simulink model "test"  (R2025b)
settings: Solver=FixedStepDiscrete  StartTime=0.0  StopTime=10.0  FixedStep=0.001  RelTol=1e-3
undefined symbols (not defined in the file): QFN64, SAMC21J18A, Timer
libraries: MCHP_Blockset x3
settings Model: SimulationMode=external  Creator=maxbo  LastModifiedBy=maxbo
settings OptimizationCC: DefaultParameterBehavior=Inlined  EnhancedBackFolding=on  PassReuseOutputArgsAs=Individual arguments  ZeroExternalMemoryAtStartup=off  ZeroInternalMemoryAtStartup=off  OptimizeBlockOrder=speed  DifferentSizesBufferReuse=on  OptimizationCustomize=off  EfficientTunableParamExpr=on
settings DebuggingCC: ParameterTunabilityLossMsg=error
settings SFSimCC: MATLABDynamicMemAlloc=off
settings RTWCC: SystemTargetFile=MCHP_ARM7_stf.tlc  TemplateMakefile=MCHP_ARM7.tmf  Toolchain=MPLAB XC32 - v5.10 for SAM & PIC32 MCUs (Microchip)  BuildConfiguration=Specify  Description=Microchip Embedded Target Cortex M7 (real-time)
settings CodeAppCC: ForceParamTrailComments=on  IgnoreCustomStorageClasses=off  OperatorAnnotations=on  SimulinkDataObjDesc=on  SFDataObjDesc=on  InsertBlockDesc=on
settings STFCustomTargetCC: SystemTargetFile=MCHP_ARM7_stf.tlc  TargetLangStandard=C99 (ISO)  MultiwordLength=256.0  ConcurrentExecutionCompliant=off  IncludeMdlTerminateFcn=off  CombineOutputUpdateFcns=on  ERTCustomFileBanners=on  SupportContinuousTime=off  RemoveResetFunc=on  MATLABClassNameForMDSCustomization=Simulink.SoftwareTarget.ERTCustomization  GRTInterface=off  BIN2HEX=xc32-bin2hex  TIMER_PRESCALER=[0 -1 -1 -1 -1]  MCHP_AUTO_FLASH=off  AssemblyListing=off  TIMER_START=[1]  PIC_REF=SAMC21J18A  RTWGenSettings_txt="s.MIPS='48000000';s.VDD_RANGE='5';s.QUARTZ='48000000';s.PLL_ENABLED='0';s.MIPS_DESIRED='48000000';s.MCLK_CPUDIV='1';s.CPU_SRC='0';s.GCLK_PCHCTRLn='[-1 -1 -1 -1 -1 -1 -1 -1 -1 -1 -1 -1 -1 -1 -1 -1 -1 -1 -1 -1 -1 -1 -1 -1 -1 -1 -1 -1 -1 -1 -1 -1 -1 -1 -1 -1 -1 -1 -1 -1 -1 -1 -1 -1 -1 -1 -1 -1]';s.OSC32KCTRL_XOSC32K_CONFIG='0';s.OSC32KCTRL_XOSC32K_ENABLE='0';s.OSC32KCTRL_XOSC32K_STARTUP='2';s.OSC32KCTRL_XOSC32K_ONDEMAND='0';s.OSC32KCTRL_XOSC32K_RUNSTDBY='1';s.OSC32KCTRL_XOSC32K_EN1K='0';s.OSC32KCTRL_XOSC32K_EN32K='1';s.OSC32KCTRL_XOSC32K_XTALEN='0';s.OSC32KCTRL_OSC32K_CONFIG='0';s.OSC32KCTRL_OSC32K_ENABLE='0';s.OSC32KCTRL_OSC32K_EN32K='0';s.OSC32KCTRL_OSC32K_EN1K='0';s.OSC32KCTRL_OSC32K_RUNSTDBY='0';s.OSC32KCTRL_OSC32K_ONDEMAND='0';s.OSC32KCTRL_OSC32K_WRTLOCK='0';s.OSC32KCTRL_OSC32K_STARTUP_CYCLEx='-1';s.OSCULP32K_CONFIG='0';s.OSCULP32K_CALIB_ENABLE='0';s.OSCULP32K_CALIB='0';s.OSCCTRL_XOSCCTRL_CONFIG='0';s.OSCCTRL_XOSCCTRL_FREQUENCY='12000000';s.OSCCTRL_XOSCCTRL_ENABLE='0';s.OSCCTRL_XOSCCTRL_STARTUP='5';s.OSCCTRL_XOSCCTRL_SWBEN='0';s.OSCCTRL_XOSCCTRL_CFDEN='0';s.OSCCTRL_XOSCCTRL_AMPGC='0';s.OSCCTRL_XOSCCTRL_GAIN='0';s.OSCCTRL_XOSCCTRL_ONDEMAND='0';s.OSCCTRL_XOSCCTRL_RUNSTDBY='1';s.OSCCTRL_XOSCCTRL_XTALEN='0';s.OSCCTRL_OSC48MCTRL_CONFIG='1';s.OSCCTRL_OSC48MCTRL_ENABLE='1';s.OSCCTRL_OSC48MCTRL_RUNSTDBY='1';s.OSCCTRL_OSC48MCTRL_ONDEMAND='0';s.OSC48MDIV_DIV='1';s.OSC48MSTUP_STARTUP='256';s.OSCCTRL_DPLLCTRL_CONFIG='0';s.OSCCTRL_DPLLCTRL_INFO_Fin='0';s.OSCCTRL_DPLLCTRL_INFO_PLLout='0';s.OSCCTRL_DPLLCTRLA_ENABLE='0';s.OSCCTRL_DPLLCTRLA_RUNSTDBY='0';s.OSCCTRL_DPLLCTRLA_ONDEMAND='0';s.OSCCTRL_DPLLRATIO_LDR='0';s.OSCCTRL_DPLLRATIO_LDRFRAC='0';s.OSCCTRL_DPLLCTRLB_FILTER_DEFAULT='0';s.OSCCTRL_DPLLCTRLB_FILTER_LBFILT='0';s.OSCCTRL_DPLLCTRLB_FILTER_HBFILT='0';s.OSCCTRL_DPLLCTRLB_FILTER_HDFILT='0';s.OSCCTRL_DPLLCTRLB_LPEN='0';s.OSCCTRL_DPLLCTRLB_WUF='0';s.OSCCTRL_DPLLCTRLB_REFCLK_XOSC32K='0';s.OSCCTRL_DPLLCTRLB_REFCLK_XOSC='0';s.OSCCTRL_DPLLCTRLB_REFCLK_GCLK='0';s.OSCCTRL_DPLLCTRLB_LTIME_DEFAULT='0';s.OSCCTRL_DPLLCTRLB_LTIME_8MS='0';s.OSCCTRL_DPLLCTRLB_LTIME_9MS='0';s.OSCCTRL_DPLLCTRLB_LTIME_10MS='0';s.OSCCTRL_DPLLCTRLB_LTIME_11MS='0';s.OSCCTRL_DPLLCTRLB_LBYPASS='0';s.OSCCTRL_DPLLCTRLB_DIV='0';s.OSCCTRL_DPLLPRESC_PRESC_DIVx='-1';s.GCLK_GENERATOR_x_CONFIG='[1 -1 -1 -1 -1 -1 -1 -1 -1]';s.GCLK_GEN_x_SOURCE='[6  0  0  0  0  0  0  0  0]';s.GCLK_GEN_x_RUNSTDBY='[1  1  1  1  1  1  1  1  1]';s.GCLK_GEN_x_DIVSEL='[0  0  0  0  0  0  0  0  0]';s.GCLK_GEN_x_OE='[0  0  0  0  0  0  0  0  0]';s.GCLK_GEN_x_OOV='[0  0  0  0  0  0  0  0  0]';s.GCLK_GEN_x_IDC='[1  1  1  1  1  1  1  1  1]';s.GCLK_GEN_x_GENEN='[1  1  1  1  1  1  1  1  1]';s.GCLK_GEN_x_DIV='[1  1  1  1  1  1  1  1  1]';s.MCLK_HSDIV='1';s.RefMasterBlk='test/Microchip Master';s.ChipIdN='[21  18  -1]';s.ChipIdL1='SAMC';s.ChipIdL2='J';s.ChipIdL3='A';s.arch3='ARM0p';s.ChipId='SAMC21J18A';s.Arch='7';s.SYS_TICK_TS_Load='47999';s.nTIMERS='5';s.nSCCP='0';s.FuseConfigTxt='/* USER_WORD_0 */\\\\n#pragma config NVMCTRL_BOOTPROT = SIZE_0BYTES\\\\n#pragma config NVMCTRL_EEPROM_SIZE = SIZE_16384BYTES\\\\n#pragma config BODVDDUSERLEVEL = 0x3F\\\\n#pragma config BODVDD_DIS = ENABLED\\\\n#pragma config BODVDD_ACTION = INT\\\\n#pragma config WDT_ENABLE = DISABLED\\\\n#pragma config WDT_ALWAYSON = DISABLED\\\\n#pragma config WDT_PER = CYC16384\\\\n/* USER_WORD_1 */\\\\n#pragma config WDT_WINDOW = CYC16384\\\\n#pragma config WDT_EWOFFSET = CYC16384\\\\n#pragma config WDT_WEN = DISABLED\\\\n#pragma config BODVDD_HYST = ENABLED\\\\n#pragma config NVMCTRL_REGION_LOCKS = 0xFFFF\\\\n';s.TimeStep_Timer='-2';s.TimeStep_SyncADC='-1';s.PINIO_REG_PMUX='[-1 -1 -1 -1 -1 -1 -1 -1 -1 -1 -1 -1 -1 -1 -1 -1 -1 -1 -1 -1 -1 -1 -1 -1 -1 -1 -1  0 -1 -1 -1 -1 -1 -1 -1 -1 -1 -1 -1 -1 -1 -1 -1 -1 -1 -1 -1 -1 -1 -1 -1 -1 -1 -1 -1 -1 -1 -1 -1 -1 -1 -1 -1 -1 -1 -1 -1 -1 -1 -1 -1 -1 -1 -1 -1 -1 -1 -1 -1 -1 -1 -1 -1 -1 -1 -1 -1 -1 -1 -1 -1 -1 -1 -1 -1 -1 -1 -1 -1 -1 -1 -1 -1 -1 -1 -1 -1 -1 -1 -1 -1 -1 -1 -1 -1 -1 -1 -1 -1 -1 -1 -1 -1 -1 -1 -1 -1 -1 -1 -1 -1 -1 -1 -1 -1 -1 -1 -1 -1 -1 -1 -1 -1 -1 -1 -1 -1 -1 -1 -1 -1 -1 -1 -1 -1 -1 -1 -1 -1 -1 -1 -1 -1 -1 -1 -1 -1 -1 -1 -1 -1 -1 -1 -1 -1 -1 -1 -1 -1 -1 -1 -1 -1 -1 -1 -1 -1 -1 -1 -1 -1 -1 -1 -1 -1 -1 -1 -1 -1 -1 -1 -1 -1 -1 -1 -1 -1 -1 -1 -1 -1 -1 -1 -1 -1 -1 -1 -1 -1 -1 -1 -1 -1 -1 -1 -1 -1 -1 -1 -1 -1 -1 -1 -1 -1 -1 -1 -1 -1 -1 -1 -1 -1 -1 -1 -1 -1 -1 -1 -1 -1 -1 -1 -1 -1 -1 -1 -1 -1 -1 -1 -1 -1 -1 -1 -1 -1 -1 -1 -1 -1 -1 -1 -1 -1 -1 -1 -1 -1 -1 -1 -1 -1 -1 -1 -1 -1 -1 -1 -1 -1 -1 -1 -1 -1 -1 -1 -1 -1 -1 -1 -1 -1 -1 -1 -1 -1 -1 -1 -1 -1 -1 -1 -1 -1 -1 -1 -1 -1 -1 -1 -1 -1 -1 -1 -1 -1 -1 -1 -1 -1 -1 -1 -1 -1 -1 -1 -1 -1 -1 -1 -1 -1 -1 -1 -1 -1 -1 -1 -1 -1 -1 -1 -1 -1 -1 -1 -1 -1 -1 -1 -1 -1 -1 -1 -1 -1 -1 -1 -1 -1 -1 -1 -1 -1 -1 -1 -1 -1 -1 -1 -1 -1 -1 -1 -1 -1 -1 -1 -1 -1 -1 -1 -1 -1 -1 -1 -1 -1 -1 -1 -1 -1 -1 -1 -1 -1 -1 -1 -1 -1 -1 -1 -1 -1 -1 -1 -1 -1 -1 -1 -1 -1 -1 -1 -1 -1 -1 -1 -1 -1 -1 -1 -1 -1 -1 -1 -1 -1 -1 -1 -1 -1 -1 -1 -1 -1 -1]';s.PINIO_DIR='[-1 -1 -1 -1 -1 -1 -1 -1 -1 -1 -1 -1 -1 -1 -1 -1 -1 -1 -1 -1 -1 -1 -1 -1 -1 -1 -1  1 -1 -1 -1 -1 -1 -1 -1 -1 -1 -1 -1 -1 -1 -1 -1 -1 -1 -1 -1 -1 -1 -1 -1 -1 -1 -1 -1 -1 -1 -1 -1 -1 -1 -1 -1 -1 -1 -1 -1 -1 -1 -1 -1 -1 -1 -1 -1 -1 -1 -1 -1 -1 -1 -1 -1 -1 -1 -1 -1 -1 -1 -1 -1 -1 -1 -1 -1 -1 -1 -1 -1 -1 -1 -1 -1 -1 -1 -1 -1 -1 -1 -1 -1 -1 -1 -1 -1 -1 -1 -1 -1 -1 -1 -1 -1 -1 -1 -1 -1 -1 -1 -1 -1 -1 -1 -1 -1 -1 -1 -1 -1 -1 -1 -1 -1 -1 -1 -1 -1 -1 -1 -1 -1 -1 -1 -1 -1 -1 -1 -1 -1 -1 -1 -1 -1 -1 -1 -1 -1 -1 -1 -1 -1 -1 -1 -1 -1 -1 -1 -1 -1 -1 -1 -1 -1 -1 -1 -1 -1 -1 -1 -1 -1 -1 -1 -1 -1 -1 -1 -1 -1 -1 -1 -1 -1 -1 -1 -1 -1 -1 -1 -1 -1 -1 -1 -1 -1 -1 -1 -1 -1 -1 -1 -1 -1 -1 -1 -1 -1 -1 -1 -1 -1 -1 -1 -1 -1 -1 -1 -1 -1 -1 -1 -1 -1 -1 -1 -1 -1 -1 -1 -1 -1 -1 -1 -1 -1 -1 -1 -1 -1 -1 -1 -1 -1 -1 -1 -1 -1 -1 -1 -1 -1 -1 -1 -1 -1 -1 -1 -1 -1 -1 -1 -1 -1 -1 -1 -1 -1 -1 -1 -1 -1 -1 -1 -1 -1 -1 -1 -1 -1 -1 -1 -1 -1 -1 -1 -1 -1 -1 -1 -1 -1 -1 -1 -1 -1 -1 -1 -1 -1 -1 -1 -1 -1 -1 -1 -1 -1 -1 -1 -1 -1 -1 -1 -1 -1 -1 -1 -1 -1 -1 -1 -1 -1 -1 -1 -1 -1 -1 -1 -1 -1 -1 -1 -1 -1 -1 -1 -1 -1 -1 -1 -1 -1 -1 -1 -1 -1 -1 -1 -1 -1 -1 -1 -1 -1 -1 -1 -1 -1 -1 -1 -1 -1 -1 -1 -1 -1 -1 -1 -1 -1 -1 -1 -1 -1 -1 -1 -1 -1 -1 -1 -1 -1 -1 -1 -1 -1 -1 -1 -1 -1 -1 -1 -1 -1 -1 -1 -1 -1 -1 -1 -1 -1 -1 -1 -1 -1 -1 -1 -1 -1 -1 -1 -1 -1 -1 -1 -1 -1 -1 -1 -1 -1 -1 -1 -1 -1 -1]';s.PINIO_DIRSET='[134217728          0          0          0          0          0          0          0          0          0          0          0          0          0]';s.PINIO_DIRCLR='[0  0  0  0  0  0  0  0  0  0  0  0  0  0]';s.PINIO_OUT='[-1 -1 -1 -1 -1 -1 -1 -1 -1 -1 -1 -1 -1 -1 -1 -1 -1 -1 -1 -1 -1 -1 -1 -1 -1 -1 -1 -1 -1 -1 -1 -1 -1 -1 -1 -1 -1 -1 -1 -1 -1 -1 -1 -1 -1 -1 -1 -1 -1 -1 -1 -1 -1 -1 -1 -1 -1 -1 -1 -1 -1 -1 -1 -1 -1 -1 -1 -1 -1 -1 -1 -1 -1 -1 -1 -1 -1 -1 -1 -1 -1 -1 -1 -1 -1 -1 -1 -1 -1 -1 -1 -1 -1 -1 -1 -1 -1 -1 -1 -1 -1 -1 -1 -1 -1 -1 -1 -1 -1 -1 -1 -1 -1 -1 -1 -1 -1 -1 -1 -1 -1 -1 -1 -1 -1 -1 -1 -1 -1 -1 -1 -1 -1 -1 -1 -1 -1 -1 -1 -1 -1 -1 -1 -1 -1 -1 -1 -1 -1 -1 -1 -1 -1 -1 -1 -1 -1 -1 -1 -1 -1 -1 -1 -1 -1 -1 -1 -1 -1 -1 -1 -1 -1 -1 -1 -1 -1 -1 -1 -1 -1 -1 -1 -1 -1 -1 -1 -1 -1 -1 -1 -1 -1 -1 -1 -1 -1 -1 -1 -1 -1 -1 -1 -1 -1 -1 -1 -1 -1 -1 -1 -1 -1 -1 -1 -1 -1 -1 -1 -1 -1 -1 -1 -1 -1 -1 -1 -1 -1 -1 -1 -1 -1 -1 -1 -1 -1 -1 -1 -1 -1 -1 -1 -1 -1 -1 -1 -1 -1 -1 -1 -1 -1 -1 -1 -1 -1 -1 -1 -1 -1 -1 -1 -1 -1 -1 -1 -1 -1 -1 -1 -1 -1 -1 -1 -1 -1 -1 -1 -1 -1 -1 -1 -1 -1 -1 -1 -1 -1 -1 -1 -1 -1 -1 -1 -1 -1 -1 -1 -1 -1 -1 -1 -1 -1 -1 -1 -1 -1 -1 -1 -1 -1 -1 -1 -1 -1 -1 -1 -1 -1 -1 -1 -1 -1 -1 -1 -1 -1 -1 -1 -1 -1 -1 -1 -1 -1 -1 -1 -1 -1 -1 -1 -1 -1 -1 -1 -1 -1 -1 -1 -1 -1 -1 -1 -1 -1 -1 -1 -1 -1 -1 -1 -1 -1 -1 -1 -1 -1 -1 -1 -1 -1 -1 -1 -1 -1 -1 -1 -1 -1 -1 -1 -1 -1 -1 -1 -1 -1 -1 -1 -1 -1 -1 -1 -1 -1 -1 -1 -1 -1 -1 -1 -1 -1 -1 -1 -1 -1 -1 -1 -1 -1 -1 -1 -1 -1 -1 -1 -1 -1 -1 -1 -1 -1 -1 -1 -1 -1 -1 -1 -1 -1 -1 -1 -1 -1 -1 -1 -1 -1 -1 -1 -1 -1 -1 -1 -1]';s.PINIO_OUTSET='[0  0  0  0  0  0  0  0  0  0  0  0  0  0]';s.PINIO_OUTCLR='[0  0  0  0  0  0  0  0  0  0  0  0  0  0]';s.PINIO_COUTINUOUS_SAMPLING='[-1 -1 -1 -1 -1 -1 -1 -1 -1 -1 -1 -1 -1 -1 -1 -1 -1 -1 -1 -1 -1 -1 -1 -1 -1 -1 -1  0 -1 -1 -1 -1 -1 -1 -1 -1 -1 -1 -1 -1 -1 -1 -1 -1 -1 -1 -1 -1 -1 -1 -1 -1 -1 -1 -1 -1 -1 -1 -1 -1 -1 -1 -1 -1 -1 -1 -1 -1 -1 -1 -1 -1 -1 -1 -1 -1 -1 -1 -1 -1 -1 -1 -1 -1 -1 -1 -1 -1 -1 -1 -1 -1 -1 -1 -1 -1 -1 -1 -1 -1 -1 -1 -1 -1 -1 -1 -1 -1 -1 -1 -1 -1 -1 -1 -1 -1 -1 -1 -1 -1 -1 -1 -1 -1 -1 -1 -1 -1 -1 -1 -1 -1 -1 -1 -1 -1 -1 -1 -1 -1 -1 -1 -1 -1 -1 -1 -1 -1 -1 -1 -1 -1 -1 -1 -1 -1 -1 -1 -1 -1 -1 -1 -1 -1 -1 -1 -1 -1 -1 -1 -1 -1 -1 -1 -1 -1 -1 -1 -1 -1 -1 -1 -1 -1 -1 -1 -1 -1 -1 -1 -1 -1 -1 -1 -1 -1 -1 -1 -1 -1 -1 -1 -1 -1 -1 -1 -1 -1 -1 -1 -1 -1 -1 -1 -1 -1 -1 -1 -1 -1 -1 -1 -1 -1 -1 -1 -1 -1 -1 -1 -1 -1 -1 -1 -1 -1 -1 -1 -1 -1 -1 -1 -1 -1 -1 -1 -1 -1 -1 -1 -1 -1 -1 -1 -1 -1 -1 -1 -1 -1 -1 -1 -1 -1 -1 -1 -1 -1 -1 -1 -1 -1 -1 -1 -1 -1 -1 -1 -1 -1 -1 -1 -1 -1 -1 -1 -1 -1 -1 -1 -1 -1 -1 -1 -1 -1 -1 -1 -1 -1 -1 -1 -1 -1 -1 -1 -1 -1 -1 -1 -1 -1 -1 -1 -1 -1 -1 -1 -1 -1 -1 -1 -1 -1 -1 -1 -1 -1 -1 -1 -1 -1 -1 -1 -1 -1 -1 -1 -1 -1 -1 -1 -1 -1 -1 -1 -1 -1 -1 -1 -1 -1 -1 -1 -1 -1 -1 -1 -1 -1 -1 -1 -1 -1 -1 -1 -1 -1 -1 -1 -1 -1 -1 -1 -1 -1 -1 -1 -1 -1 -1 -1 -1 -1 -1 -1 -1 -1 -1 -1 -1 -1 -1 -1 -1 -1 -1 -1 -1 -1 -1 -1 -1 -1 -1 -1 -1 -1 -1 -1 -1 -1 -1 -1 -1 -1 -1 -1 -1 -1 -1 -1 -1 -1 -1 -1 -1 -1 -1 -1 -1 -1 -1 -1 -1 -1 -1 -1 -1 -1 -1 -1 -1 -1 -1 -1 -1 -1]';s.PINIO_OUT_STRENGTH='[-1 -1 -1 -1 -1 -1 -1 -1 -1 -1 -1 -1 -1 -1 -1 -1 -1 -1 -1 -1 -1 -1 -1 -1 -1 -1 -1  0 -1 -1 -1 -1 -1 -1 -1 -1 -1 -1 -1 -1 -1 -1 -1 -1 -1 -1 -1 -1 -1 -1 -1 -1 -1 -1 -1 -1 -1 -1 -1 -1 -1 -1 -1 -1 -1 -1 -1 -1 -1 -1 -1 -1 -1 -1 -1 -1 -1 -1 -1 -1 -1 -1 -1 -1 -1 -1 -1 -1 -1 -1 -1 -1 -1 -1 -1 -1 -1 -1 -1 -1 -1 -1 -1 -1 -1 -1 -1 -1 -1 -1 -1 -1 -1 -1 -1 -1 -1 -1 -1 -1 -1 -1 -1 -1 -1 -1 -1 -1 -1 -1 -1 -1 -1 -1 -1 -1 -1 -1 -1 -1 -1 -1 -1 -1 -1 -1 -1 -1 -1 -1 -1 -1 -1 -1 -1 -1 -1 -1 -1 -1 -1 -1 -1 -1 -1 -1 -1 -1 -1 -1 -1 -1 -1 -1 -1 -1 -1 -1 -1 -1 -1 -1 -1 -1 -1 -1 -1 -1 -1 -1 -1 -1 -1 -1 -1 -1 -1 -1 -1 -1 -1 -1 -1 -1 -1 -1 -1 -1 -1 -1 -1 -1 -1 -1 -1 -1 -1 -1 -1 -1 -1 -1 -1 -1 -1 -1 -1 -1 -1 -1 -1 -1 -1 -1 -1 -1 -1 -1 -1 -1 -1 -1 -1 -1 -1 -1 -1 -1 -1 -1 -1 -1 -1 -1 -1 -1 -1 -1 -1 -1 -1 -1 -1 -1 -1 -1 -1 -1 -1 -1 -1 -1 -1 -1 -1 -1 -1 -1 -1 -1 -1 -1 -1 -1 -1 -1 -1 -1 -1 -1 -1 -1 -1 -1 -1 -1 -1 -1 -1 -1 -1 -1 -1 -1 -1 -1 -1 -1 -1 -1 -1 -1 -1 -1 -1 -1 -1 -1 -1 -1 -1 -1 -1 -1 -1 -1 -1 -1 -1 -1 -1 -1 -1 -1 -1 -1 -1 -1 -1 -1 -1 -1 -1 -1 -1 -1 -1 -1 -1 -1 -1 -1 -1 -1 -1 -1 -1 -1 -1 -1 -1 -1 -1 -1 -1 -1 -1 -1 -1 -1 -1 -1 -1 -1 -1 -1 -1 -1 -1 -1 -1 -1 -1 -1 -1 -1 -1 -1 -1 -1 -1 -1 -1 -1 -1 -1 -1 -1 -1 -1 -1 -1 -1 -1 -1 -1 -1 -1 -1 -1 -1 -1 -1 -1 -1 -1 -1 -1 -1 -1 -1 -1 -1 -1 -1 -1 -1 -1 -1 -1 -1 -1 -1 -1 -1 -1 -1 -1 -1 -1 -1 -1 -1 -1 -1 -1 -1 -1]';s.PINIO_PULLEN='[-1 -1 -1 -1 -1 -1 -1 -1 -1 -1 -1 -1 -1 -1 -1 -1 -1 -1 -1 -1 -1 -1 -1 -1 -1 -1 -1  0 -1 -1 -1 -1 -1 -1 -1 -1 -1 -1 -1 -1 -1 -1 -1 -1 -1 -1 -1 -1 -1 -1 -1 -1 -1 -1 -1 -1 -1 -1 -1 -1 -1 -1 -1 -1 -1 -1 -1 -1 -1 -1 -1 -1 -1 -1 -1 -1 -1 -1 -1 -1 -1 -1 -1 -1 -1 -1 -1 -1 -1 -1 -1 -1 -1 -1 -1 -1 -1 -1 -1 -1 -1 -1 -1 -1 -1 -1 -1 -1 -1 -1 -1 -1 -1 -1 -1 -1 -1 -1 -1 -1 -1 -1 -1 -1 -1 -1 -1 -1 -1 -1 -1 -1 -1 -1 -1 -1 -1 -1 -1 -1 -1 -1 -1 -1 -1 -1 -1 -1 -1 -1 -1 -1 -1 -1 -1 -1 -1 -1 -1 -1 -1 -1 -1 -1 -1 -1 -1 -1 -1 -1 -1 -1 -1 -1 -1 -1 -1 -1 -1 -1 -1 -1 -1 -1 -1 -1 -1 -1 -1 -1 -1 -1 -1 -1 -1 -1 -1 -1 -1 -1 -1 -1 -1 -1 -1 -1 -1 -1 -1 -1 -1 -1 -1 -1 -1 -1 -1 -1 -1 -1 -1 -1 -1 -1 -1 -1 -1 -1 -1 -1 -1 -1 -1 -1 -1 -1 -1 -1 -1 -1 -1 -1 -1 -1 -1 -1 -1 -1 -1 -1 -1 -1 -1 -1 -1 -1 -1 -1 -1 -1 -1 -1 -1 -1 -1 -1 -1 -1 -1 -1 -1 -1 -1 -1 -1 -1 -1 -1 -1 -1 -1 -1 -1 -1 -1 -1 -1 -1 -1 -1 -1 -1 -1 -1 -1 -1 -1 -1 -1 -1 -1 -1 -1 -1 -1 -1 -1 -1 -1 -1 -1 -1 -1 -1 -1 -1 -1 -1 -1 -1 -1 -1 -1 -1 -1 -1 -1 -1 -1 -1 -1 -1 -1 -1 -1 -1 -1 -1 -1 -1 -1 -1 -1 -1 -1 -1 -1 -1 -1 -1 -1 -1 -1 -1 -1 -1 -1 -1 -1 -1 -1 -1 -1 -1 -1 -1 -1 -1 -1 -1 -1 -1 -1 -1 -1 -1 -1 -1 -1 -1 -1 -1 -1 -1 -1 -1 -1 -1 -1 -1 -1 -1 -1 -1 -1 -1 -1 -1 -1 -1 -1 -1 -1 -1 -1 -1 -1 -1 -1 -1 -1 -1 -1 -1 -1 -1 -1 -1 -1 -1 -1 -1 -1 -1 -1 -1 -1 -1 -1 -1 -1 -1 -1 -1 -1 -1 -1 -1 -1 -1 -1 -1 -1 -1 -1 -1 -1 -1]';s.PINIO_INPUT_ENABLE='[-1 -1 -1 -1 -1 -1 -1 -1 -1 -1 -1 -1 -1 -1 -1 -1 -1 -1 -1 -1 -1 -1 -1 -1 -1 -1 -1  0 -1 -1 -1 -1 -1 -1 -1 -1 -1 -1 -1 -1 -1 -1 -1 -1 -1 -1 -1 -1 -1 -1 -1 -1 -1 -1 -1 -1 -1 -1 -1 -1 -1 -1 -1 -1 -1 -1 -1 -1 -1 -1 -1 -1 -1 -1 -1 -1 -1 -1 -1 -1 -1 -1 -1 -1 -1 -1 -1 -1 -1 -1 -1 -1 -1 -1 -1 -1 -1 -1 -1 -1 -1 -1 -1 -1 -1 -1 -1 -1 -1 -1 -1 -1 -1 -1 -1 -1 -1 -1 -1 -1 -1 -1 -1 -1 -1 -1 -1 -1 -1 -1 -1 -1 -1 -1 -1 -1 -1 -1 -1 -1 -1 -1 -1 -1 -1 -1 -1 -1 -1 -1 -1 -1 -1 -1 -1 -1 -1 -1 -1 -1 -1 -1 -1 -1 -1 -1 -1 -1 -1 -1 -1 -1 -1 -1 -1 -1 -1 -1 -1 -1 -1 -1 -1 -1 -1 -1 -1 -1 -1 -1 -1 -1 -1 -1 -1 -1 -1 -1 -1 -1 -1 -1 -1 -1 -1 -1 -1 -1 -1 -1 -1 -1 -1 -1 -1 -1 -1 -1 -1 -1 -1 -1 -1 -1 -1 -1 -1 -1 -1 -1 -1 -1 -1 -1 -1 -1 -1 -1 -1 -1 -1 -1 -1 -1 -1 -1 -1 -1 -1 -1 -1 -1 -1 -1 -1 -1 -1 -1 -1 -1 -1 -1 -1 -1 -1 -1 -1 -1 -1 -1 -1 -1 -1 -1 -1 -1 -1 -1 -1 -1 -1 -1 -1 -1 -1 -1 -1 -1 -1 -1 -1 -1 -1 -1 -1 -1 -1 -1 -1 -1 -1 -1 -1 -1 -1 -1 -1 -1 -1 -1 -1 -1 -1 -1 -1 -1 -1 -1 -1 -1 -1 -1 -1 -1 -1 -1 -1 -1 -1 -1 -1 -1 -1 -1 -1 -1 -1 -1 -1 -1 -1 -1 -1 -1 -1 -1 -1 -1 -1 -1 -1 -1 -1 -1 -1 -1 -1 -1 -1 -1 -1 -1 -1 -1 -1 -1 -1 -1 -1 -1 -1 -1 -1 -1 -1 -1 -1 -1 -1 -1 -1 -1 -1 -1 -1 -1 -1 -1 -1 -1 -1 -1 -1 -1 -1 -1 -1 -1 -1 -1 -1 -1 -1 -1 -1 -1 -1 -1 -1 -1 -1 -1 -1 -1 -1 -1 -1 -1 -1 -1 -1 -1 -1 -1 -1 -1 -1 -1 -1 -1 -1 -1 -1 -1 -1 -1 -1 -1 -1 -1 -1 -1 -1 -1 -1 -1 -1 -1]';s.PINIO_PMUX_ENABLE='[1  1  1  1  1  1  1  1  1  1  1  1  1  1  1  1  1  1  1  1  1  1  1  1  1  1  1  0  1  1  1  1  1  1  1  1  1  1  1  1  1  1  1  1  1  1  1  1  1  1  1  1  1  1  1  1  1  1  1  1  1  1  1  1  1  1  1  1  1  1  1  1  1  1  1  1  1  1  1  1  1  1  1  1  1  1  1  1  1  1  1  1  1  1  1  1  1  1  1  1  1  1  1  1  1  1  1  1  1  1  1  1  1  1  1  1  1  1  1  1  1  1  1  1  1  1  1  1  1  1  1  1  1  1  1  1  1  1  1  1  1  1  1  1  1  1  1  1  1  1  1  1  1  1  1  1  1  1  1  1  1  1  1  1  1  1  1  1  1  1  1  1  1  1  1  1  1  1  1  1  1  1  1  1  1  1  1  1  1  1  1  1  1  1  1  1  1  1  1  1  1  1  1  1  1  1  1  1  1  1  1  1  1  1  1  1  1  1  1  1  1  1  1  1  1  1  1  1  1  1  1  1  1  1  1  1  1  1  1  1  1  1  1  1  1  1  1  1  1  1  1  1  1  1  1  1  1  1  1  1  1  1  1  1  1  1  1  1  1  1  1  1  1  1  1  1  1  1  1  1  1  1  1  1  1  1  1  1  1  1  1  1  1  1  1  1  1  1  1  1  1  1  1  1  1  1  1  1  1  1  1  1  1  1  1  1  1  1  1  1  1  1  1  1  1  1  1  1  1  1  1  1  1  1  1  1  1  1  1  1  1  1  1  1  1  1  1  1  1  1  1  1  1  1  1  1  1  1  1  1  1  1  1  1  1  1  1  1  1  1  1  1  1  1  1  1  1  1  1  1  1  1  1  1  1  1  1  1  1  1  1  1  1  1  1  1  1  1  1  1  1  1  1  1  1  1  1  1  1  1  1  1  1  1  1  1  1  1  1  1  1  1  1  1  1  1  1  1  1  1  1  1  1  1  1  1  1  1  1  1  1  1  1  1  1  1  1  1]';s.MASTER_BusyFlag='-1';s.POWERSAVE='0';s.UART_TX_IMPLEMENTATION='[2  4  0  0  2  0  0  0]';s.UART_RX_IMPLEMENTATION='[2  2  0  0  2  0  0  0]';s.UART_TX_DMACHANNEL='[0  0 -1 -1  0]';s.UART_RX_DMACHANNEL='[0  0 -1 -1  0]';s.DMA_Channel_active='[0  1]';s.DMA_active_num_channels='[1]';s.UART_HALF_DUPLEX_MODE='[0  0  0  0  0]';s.UART_TX_THREAD_PROTECTION='[9  9  0  0  9]';"  AR1=xc32-ar  OBJDUMP=xc32-objdump  GCCPATH=C:/PROGRA~1/MICROC~1/xc32/v5.10/bin  MCHP_XCP_MemoryBlockParameters=[-1 8]  OPTIM_GCC=-O2 -g  HOST_PLATFORM=PC  MCHP_MULTITHREAD_COMPILATION=on  GCC1=xc32-gcc.exe  LDFLAGS='--report-mem,-Map=$(PRODUCT_NAME).map,-cref,--memorysummary,memoryfile.xml'  MCHP_CompiledTime_ModelSampleTimes_Txt=s.Value=reshape([0.001 0],1,2);s.Description='Discrete 1';s.ColorRGBValue=reshape(MCHP_Fun.Hex2num('[3FF0000000000000 3FD1515151515151 3FCD1D1D1D1D1D1D]'),1,3);s.Annotation='D1';s.TID=0;s.Owner=[];s.ComponentSampleTimes=[];  EXTMODE_DATA_UPLOAD=off  TIMER_PERIOD=[65535]  ProduceHexOutput=off
settings ERTTargetCC: ERTSrcFileBannerTemplate=MCHP_dsPIC_code_template.cgt  ERTHdrFileBannerTemplate=MCHP_dsPIC_code_template.cgt  ERTDataSrcFileTemplate=MCHP_dsPIC_code_template.cgt  ERTDataHdrFileTemplate=MCHP_dsPIC_code_template.cgt  ERTCustomFileTemplate=MCHP_main.tlc  TargetLangStandard=C99 (ISO)  ParMdlRefBuildCompliant=off  CompOptLevelCompliant=off  ConcurrentExecutionCompliant=off  IncludeMdlTerminateFcn=off  SupportNonInlinedSFcns=on  ModelStepFunctionPrototypeControlCompliant=off  CPPClassGenCompliant=off  UseToolchainInfoCompliant=off

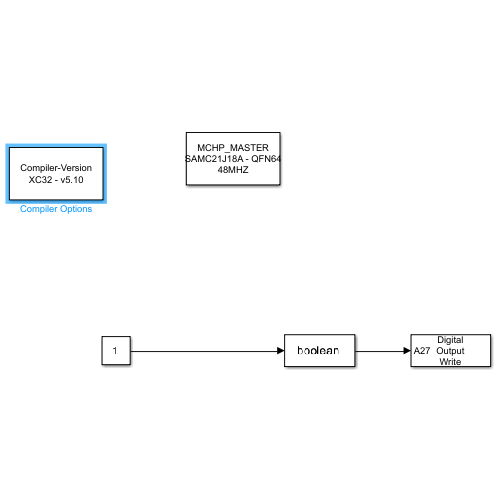
[thumbnail: Simulink's stored preview of the top-level diagram]
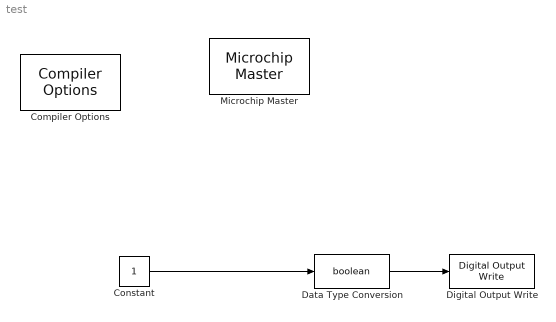
== system test ==
  Compiler Options : MCHP_Blockset/System Configuration/Compiler Options  Priority=1  LATEST_CMPLR=on  COMP_LIST_TXT=XC32 - v5.10  DFP_LIST_TXT=Update DFP list  CMSIS_DSP_TXT=Not used  USE_64BIT_DOUBLE=off  MCHP_MULTITHREAD_COMPILATION=on  UseCustom_LinkerScript=off  MCHP_MASTERLINK=test/Microchip Master  OPTIMIZATION_LEVEL=2  MPLAB_LINKLIB=default  MPLAB_LINKLIB1=fast floating-point math  CodeReplacement_TXT=None  OPTIMIZATION_FLTO=off  OPTIMIZATION_REORDER=off  OPTIMIZATION_ASM_REORDER=off  UNROLL_LOOPS=off  PROCEDURAL_ABSTRACTION=off  CONSERVE_STACK=off  GC_SECTIONS=None  MCODE=is less than 32768 (faster)  MCONST=in data memory  MDATA=Use only memory below address 8192 (faster)  MSCALAR=Use only memory below address 8192 (faster)  MLARGEARRAY=off  MAGGREGATE=off  HEAP_SIZE=0  OMF=elf  DEBUG_INFO=on  MCHP_STACK_USAGE=off  GCC_STACK_USAGE=off  ProduceHexOutput=off  AssemblyListing=off  SaveTemps=off  NO_EDS_WARN=on  PRINT_STATISTICS=off
      settings: SourceProductName=MPLAB Device Blocks for Simulink
  Constant : Constant  SampleTime=0.001
  Data Type Conversion : DataTypeConversion  OutDataTypeStr=boolean  SaturateOnIntegerOverflow=off  RndMeth=Floor
  Digital Output Write : MCHP_Blockset/Digital IO/Digital Output Write  PORT_TXT="A   [ 0  1  2  3  4  5  6  7  8  9  10  11  12  13  14  15  16  17  18  19  20  21  22  23  24  25  27  28  30  31 ]"  PIN=27  INIT_VALUE=-1  PACK=off  OUTPUT_PIN_MODE=Push-Pull (default)  SIMULTANEOUS=off  ORDERING=None  SampleTime=-1  MCHP_PORT={Digital Out}{DOU}1:1:A27;  MCHP_MASTERLINK=test/Microchip Master
      settings: SourceProductName=MPLAB Device Blocks for Simulink
  Microchip Master : MCHP_Blockset/System Configuration/Microchip Master  Priority=1  PICREF=SAMC21J18A - QFN64  TIMESTEP_REF="Timer  ( 0.001s )"  BUSYFLAG=Dynamic Options  BUSYFLAG_TXT=None  VDD_range=Dynamic Options  VDD_range_TXT=4.5V to 5.5V  PWRTEN=Not used  BOREN=Enabled  BODENV=2.7V  BORV=Not used  FPWRT=128ms  DSBOREN=Disable ZPBOR during Deep Sleep Mode  DSLPBOR=Not used  MCLRE=Enabled  SMCLR=MCLR pin generates a normal system Reset  PMDL1WAY=Allow only one reconfiguration  RSTPRI=Device will obtain reset instruction from Primary flash  TEMP=Not used  SOSCSRC=Not used  SOSCSEL=Not used  IOL1WAY=Allow multiple reconfigurations  ALTVREF=Not used  DISUVREG=Not used  DSSWEN=Not used  LPCFG=Not used  RTCBAT=Not used  VBTBOR=Not used  WUTSEL=Not used  POWERSAVE=off  FNOSC=Internal Fast RC (FRC)  FPR=ECIO w/ PLL 16x  FOSFPR=HS3 w/PLL 16x  FOS=Primary Oscillator  FRANGE=High Range  OSCILLATOR_SELECT=Internal 48MHz Oscillator  OSCILLATOR_SELECT_spd=Internal 48MHz Oscillator  QUARTZ=48e6  QUARTZ_spd=48e6  POSCGAIN=2x gain setting  POSCBOOST=Boost the kick start of the oscillator  SOSCGAIN=2x gain setting  SOSCBOOST=Boost the kick start of the oscillator  ACTIV_PLL=off  ACTIV_PLL_spd=off  MIPS_DESIRED=7370000  MIPS_DESIRED_spd=7370000  CPUDIV=Divide by 1  FPLLMUL=Not used  FPLLIDIV=8x Divider  POSCFREQ=Not used  POSCMD=Primary Oscillator Disabled  POSCMOD=Primary osc disabled  MIPS=48 * 1e6  ACLKCON=Optimized for PWM resolution & ADC conversion speed  ACLKCON_spd=Optimized for PWM resolution & ADC conversion speed  FPLLODIV=32x Divider  PLLKEN=Clock switch to PLL source will wait until the PLL lock signal is valid  FCKSM=Both Clock switching and Fail-safe Clock Monitor are disabled  FCKSMEN=Sw Disabled; Mon Disabled  IESO=Start up with FRC; then switch  DSWDTPS=1:2^36  FWDTEN=Disable  FWDTWINSZ=Window size is 25%  FWPSA=1:512  FWPSA0=1:128  FWPSB=1:16  WDT=Disable  WDTPOST=1:32768  WDTPRE=1:128  WDTPS=1:1048576  WINDIS=Watchdog Timer in Non-Window mode  WWDTEN=Window mode  DSWDTEN=Disable DSWDT during Deep Sleep Mode  DSWDTOSC=Select LPRC as DSWDT Reference clock  FWDT_RCLKSEL=WDT Run Mode uses BFRC:256  FWDT_RWDTPS=1:2147483648  FWDT_SWDTMPS=1:2147483648  FWDT_WDTEN=Enable  FWDT_WDTRSTEN=WDT event generates a reset  FWDT_WDTWIN=WDT Window is 25% of WDT period  FWDT_WINEN=Not used  FPBDIV=Not used  FSOSCEN=Disable Secondary Oscillator  LPRCSEL=Not used  OSCIOFCN=Not used  OSCIOFNC=general purpose digital I/O pin  LVRCFG=Not used  PLL_96MHZ=Not used  PLL96MHZ=Not used  PLLDIV=Not used  WDTCLK=Not used  WDTCMX=Not used  WDTWIN=Watchdog Window is 25% of WDT period  XTCFG=24-32 MHz crystals  XTBST=Boost the kick-start  APL=Aux Flash Code protect is disabled  APLK=Aux Flash Write Protection or Code Protection is Enabled  AWRP=Auxiliary program memory is not write-protected  BSS=No Boot program Flash segment  BWP=Not used  BWRP=Boot Segment may be written  CP=Protection Disabled  EBS=No Boot EEPROM  ESS=No Segment Data EEPROM  GCP=General Segment Code protect is Disabled  GSS=General Segment Code protect is Disabled  GSS0=Not used  GSSK=General Segment Write Protection or Code Protection is Enabled  GWRP=General Segment may be written  PWP=Not used  RBS=No Boot RAM  RSS=No Secure RAM  SSS=No Secure Segment  SWRP=Secure segment may be written  WPCFG=Not used  WPDIS=Not used  WPEND=Not used  WPFP=Not used  ICESEL=Communicate on PGEC1/PGED1  ICS=Communicate on PGEC1 and PGED1  JTAGEN=Disable  FICD_JTAGEN=Disable  COE=Not used  RES=Not used  DEBUG=Debugger is disabled  BACKBUG=Not used  BKBUG=Not used  ALTI2C=I2C mapped to SDA1/SCL1 pins  ALTI2C1=SDA1/SCK1 pins are selected as the I/O pins for I2C1  ALTI2C2=SDA2/SCK2 pins are selected as the I/O pins for I2C2  ALTI2C3=I2C3 mapped to SDA3/SCL3 pins  FDEVOPT1_ALTI2C1=Not used  FDEVOPT1_ALTI2C2=Not used  FDEVOPT1_SPI2MAPDIS=Not used  FDEVOPT_ALTI2C1=Primary I2C1 pins are used  FDEVOPT_ALTI2C2=Primary I2C2 pins are used  FDEVOPT_ALTI2C3=Primary I2C3 pins are used  FDEVOPT_SPI2PIN=SPI2 pins are selected by peripheral pin selection feature  ALTQIO=QEA1; QEB1; INDX1 are selected as inputs to QEI1  ALTSS1=SS1A is selected as the I/O pin for SPI1  CMPPOL0=Hysteresis is applied to falling edge  CMPPOL1=Hysteresis is applied to falling edge  FCANIO=Not used  FETHIO=Default Ethernet I/O  FMIIEN=MII Enabled  FSRSSEL=Not used  FUSBIDIO=Controlled by the USB Module  FVBUSONIO=Not used  HPOL=PWM module high side output pins have active-high output polarity  HYST0=45 mV Hysteresis  HYST1=45 mV Hysteresis  I2C1SEL=Not used  LPOL=PWM module low side output pins have active-high output polarity  PWMPIN=PWM module pins controlled by PORT register at device Reset  RTCOSC=Not used  UPLLEN=USB PLL Disabled  UPLLIDIV=Not used  ATMOD8=Not used  ALTPMP=Not used  I2C2SEL=Not used  ALTADREF=Not used  ALTCVREF=Not used  PWMLOCK=PWM registers may be written without key sequence  INT_PRIORITY_DMA=0  MCHP_TIMER_RESULT=[1 3684 ]  MCHP_PLLRegisters=[-1 -1 -1 -1 -1]  MCHPVAR=MCHP.id.name='SAMC21J18A';MCHP.id.N=reshape([21 18 -1],1,3);MCHP.id.L=reshape({ 'SAMC','J','A'},1,3);MCHP.id.maskset=' ';MCHP.id.dos=' ';MCHP.id.ds=' ';MCHP.id.archTxt=' ';MCHP.id.clonedfrom=' ';MCHP.id.Arch=7;MCHP.id.pinout={ 'QFN64'};MCHP.Rx=reshape([1 61 2 62 3 63 4 64 13 5 14 6 15 9 16 10 17 11 18 12 19 23 20 24 29 25 30 26 31 27 32 28 35 39 36 40 37 -1 38 -1 41 -1 42 -1 43 49 44 50 45 -1 46 -1 -1 -1 51 -1 53 -1 -1 -1 57 59 58 60],2,32);MCHP.memory.FLASH.size=262144;MCHP.memory.OTP5.size=8;MCHP.memory.TEMP_LOG.size=8;MCHP.memory.USER_PAGE.size=256;MCHP.memory.RWW.size=8192;MCHP.memory.HSRAM.size=32768;MCHP.memory.HPB0.size=16384;MCHP.memory.HPB1.size=65536;MCHP.memory.HPB2.size=32768;MCHP.memory.DIVAS.size=32;MCHP.memory.PPB.size=1048576;MCHP.memory.SCS.size=4096;MCHP.memory.PERIPHERALS.size=MCHP_Fun.Hex2num('41C0000000000000');MCHP.module.MCLK_OSCCTRL_OSC32KCTRL_PAC_SUPC.PID=0;MCHP.module.MCLK_OSCCTRL_OSC32KCTRL_PAC_SUPC.vector='SYSTEM';MCHP.module.WDT.PID=1;MCHP.module.WDT.vector='WDT';MCHP.module.RTC.PID=2;MCHP.module.RTC.vector='RTC';MCHP.module.EIC.PID=3;MCHP.module.EIC.vector='EIC';MCHP.module.EIC.pin.EXTINT0.txt=reshape({ 'PA16','PB00','PB16','PA00'},1,4);MCHP.module.EIC.pin.EXTINT0.Rx_idx=reshape([16 32 48 0],1,4);MCHP.module.EIC.pin.EXTINT0.ABCD=reshape([0 0 0 0],1,4);MCHP.module.EIC.pin.EXTINT1.txt=reshape({ 'PA17','PB01','PB17','PA01'},1,4);MCHP.module.EIC.pin.EXTINT1.Rx_idx=reshape([17 33 49 1],1,4);MCHP.module.EIC.pin.EXTINT1.ABCD=reshape([0 0 0 0],1,4);MCHP.module.EIC.pin.EXTINT2.txt=reshape({ 'PA02','PA18','PB02'},1,3);MCHP.module.EIC.pin.EXTINT2.Rx_idx=reshape([2 18 34],1,3);MCHP.module.EIC.pin.EXTINT2.ABCD=reshape([0 0 0],1,3);MCHP.module.EIC.pin.EXTINT3.txt=reshape({ 'PA03','PA19','PB03'},1,3);MCHP.module.EIC.pin.EXTINT3.Rx_idx=reshape([3 19 35],1,3);MCHP.module.EIC.pin.EXTINT3.ABCD=reshape([0 0 0],1,3);MCHP.module.EIC.pin.EXTINT4.txt=reshape({ 'PA04','PA20','PB04'},1,3);MCHP.module.EIC.pin.EXTINT4.Rx_idx=reshape([4 20 36],1,3);MCHP.module.EIC.pin.EXTINT4.ABCD=reshape([0 0 0],1,3);MCHP.module.EIC.pin.EXTINT5.txt=reshape({ 'PA05','PA21','PB05'},1,3);MCHP.module.EIC.pin.EXTINT5.Rx_idx=reshape([5 21 37],1,3);MCHP.module.EIC.pin.EXTINT5.ABCD=reshape([0 0 0],1,3);MCHP.module.EIC.pin.EXTINT6.txt=reshape({ 'PA06','PA22','PB06','PB22'},1,4);MCHP.module.EIC.pin.EXTINT6.Rx_idx=reshape([6 22 38 54],1,4);MCHP.module.EIC.pin.EXTINT6.ABCD=reshape([0 0 0 0],1,4);MCHP.module.EIC.pin.EXTINT7.txt=reshape({ 'PA07','PA23','PB07','PB23'},1,4);MCHP.module.EIC.pin.EXTINT7.Rx_idx=reshape([7 23 39 55],1,4);MCHP.module.EIC.pin.EXTINT7.ABCD=reshape([0 0 0 0],1,4);MCHP.module.EIC.pin.EXTINT8.txt=reshape({ 'PB08','PA28'},1,2);MCHP.module.EIC.pin.EXTINT8.Rx_idx=reshape([40 28],1,2);MCHP.module.EIC.pin.EXTINT8.ABCD=reshape([0 0],1,2);MCHP.module.EIC.pin.EXTINT9.txt=reshape({ 'PA09','PB09'},1,2);MCHP.module.EIC.pin.EXTINT9.Rx_idx=reshape([9 41],1,2);MCHP.module.EIC.pin.EXTINT9.ABCD=reshape([0 0],1,2);MCHP.module.EIC.pin.EXTINT10.txt=reshape({ 'PA10','PA30','PB10'},1,3);MCHP.module.EIC.pin.EXTINT10.Rx_idx=reshape([10 30 42],1,3);MCHP.module.EIC.pin.EXTINT10.ABCD=reshape([0 0 0],1,3);MCHP.module.EIC.pin.EXTINT11.txt=reshape({ 'PA11','PA31','PB11'},1,3);MCHP.module.EIC.pin.EXTINT11.Rx_idx=reshape([11 31 43],1,3);MCHP.module.EIC.pin.EXTINT11.ABCD=reshape([0 0 0],1,3);MCHP.module.EIC.pin.EXTINT12.txt=reshape({ 'PA12','PA24','PB12'},1,3);MCHP.module.EIC.pin.EXTINT12.Rx_idx=reshape([12 24 44],1,3);MCHP.module.EIC.pin.EXTINT12.ABCD=reshape([0 0 0],1,3);MCHP.module.EIC.pin.EXTINT13.txt=reshape({ 'PA13','PA25','PB13'},1,3);MCHP.module.EIC.pin.EXTINT13.Rx_idx=reshape([13 25 45],1,3);MCHP.module.EIC.pin.EXTINT13.ABCD=reshape([0 0 0],1,3);MCHP.module.EIC.pin.EXTINT14.txt=reshape({ 'PB14','PB30','PA14'},1,3);MCHP.module.EIC.pin.EXTINT14.Rx_idx=reshape([46 62 14],1,3);MCHP.module.EIC.pin.EXTINT14.ABCD=reshape([0 0 0],1,3);MCHP.module.EIC.pin.EXTINT15.txt=reshape({ 'PA27','PB15','PB31','PA15'},1,4);MCHP.module.EIC.pin.EXTINT15.Rx_idx=reshape([27 47 63 15],1,4);MCHP.module.EIC.pin.EXTINT15.ABCD=reshape([0 0 0 0],1,4);MCHP.module.EIC.pin.NMI.txt={ 'PA08'};MCHP.module.EIC.pin.NMI.Rx_idx=8;MCHP.module.EIC.pin.NMI.ABCD=0;MCHP.module.FREQM.PID=4;MCHP.module.FREQM.vector='FREQM';MCHP.module.TSENS.PID=5;MCHP.module.TSENS.vector='TSENS';MCHP.module.NVMCTRL.PID=6;MCHP.module.NVMCTRL.vector='NVMCTRL';MCHP.module.DMAC.PID=7;MCHP.module.DMAC.vector='DMAC';MCHP.module.EVSYS.PID=8;MCHP.module.EVSYS.vector='EVSYS';MCHP.module.SERCOM0.PID=9;MCHP.module.SERCOM0.vector='SERCOM0';MCHP.module.SERCOM0.pin.PAD0.txt=reshape({ 'PA04','PA08'},1,2);MCHP.module.SERCOM0.pin.PAD0.Rx_idx=reshape([4 8],1,2);MCHP.module.SERCOM0.pin.PAD0.ABCD=reshape([3 2],1,2);MCHP.module.SERCOM0.pin.PAD1.txt=reshape({ 'PA05','PA09'},1,2);MCHP.module.SERCOM0.pin.PAD1.Rx_idx=reshape([5 9],1,2);MCHP.module.SERCOM0.pin.PAD1.ABCD=reshape([3 2],1,2);MCHP.module.SERCOM0.pin.PAD2.txt=reshape({ 'PA06','PA10'},1,2);MCHP.module.SERCOM0.pin.PAD2.Rx_idx=reshape([6 10],1,2);MCHP.module.SERCOM0.pin.PAD2.ABCD=reshape([3 2],1,2);MCHP.module.SERCOM0.pin.PAD3.txt=reshape({ 'PA07','PA11'},1,2);MCHP.module.SERCOM0.pin.PAD3.Rx_idx=reshape([7 11],1,2);MCHP.module.SERCOM0.pin.PAD3.ABCD=reshape([3 2],1,2);MCHP.module.SERCOM1.PID=10;MCHP.module.SERCOM1.vector='SERCOM1';MCHP.module.SERCOM1.pin.PAD0.txt=reshape({ 'PA16','PA00'},1,2);MCHP.module.SERCOM1.pin.PAD0.Rx_idx=reshape([16 0],1,2);MCHP.module.SERCOM1.pin.PAD0.ABCD=reshape([2 3],1,2);MCHP.module.SERCOM1.pin.PAD1.txt=reshape({ 'PA17','PA01'},1,2);MCHP.module.SERCOM1.pin.PAD1.Rx_idx=reshape([17 1],1,2);MCHP.module.SERCOM1.pin.PAD1.ABCD=reshape([2 3],1,2);MCHP.module.SERCOM1.pin.PAD2.txt=reshape({ 'PA30','PA18'},1,2);MCHP.module.SERCOM1.pin.PAD2.Rx_idx=reshape([30 18],1,2);MCHP.module.SERCOM1.pin.PAD2.ABCD=reshape([3 2],1,2);MCHP.module.SERCOM1.pin.PAD3.txt=reshape({ 'PA31','PA19'},1,2);MCHP.module.SERCOM1.pin.PAD3.Rx_idx=reshape([31 19],1,2);MCHP.module.SERCOM1.pin.PAD3.ABCD=reshape([3 2],1,2);MCHP.module.SERCOM2.PID=11;MCHP.module.SERCOM2.vector='SERCOM2';MCHP.module.SERCOM2.pin.PAD0.txt=reshape({ 'PA08','PA12'},1,2);MCHP.module.SERCOM2.pin.PAD0.Rx_idx=reshape([8 12],1,2);MCHP.module.SERCOM2.pin.PAD0.ABCD=reshape([3 2],1,2);MCHP.module.SERCOM2.pin.PAD1.txt=reshape({ 'PA09','PA13'},1,2);MCHP.module.SERCOM2.pin.PAD1.Rx_idx=reshape([9 13],1,2);MCHP.module.SERCOM2.pin.PAD1.ABCD=reshape([3 2],1,2);MCHP.module.SERCOM2.pin.PAD2.txt=reshape({ 'PA10','PA14'},1,2);MCHP.module.SERCOM2.pin.PAD2.Rx_idx=reshape([10 14],1,2);MCHP.module.SERCOM2.pin.PAD2.ABCD=reshape([3 2],1,2);MCHP.module.SERCOM2.pin.PAD3.txt=reshape({ 'PA11','PA15'},1,2);MCHP.module.SERCOM2.pin.PAD3.Rx_idx=reshape([11 15],1,2);MCHP.module.SERCOM2.pin.PAD3.ABCD=reshape([3 2],1,2);MCHP.module.SERCOM3.PID=12;MCHP.module.SERCOM3.vector='SERCOM3';MCHP.module.SERCOM3.pin.PAD0.txt=reshape({ 'PA16','PA22'},1,2);MCHP.module.SERCOM3.pin.PAD0.Rx_idx=reshape([16 22],1,2);MCHP.module.SERCOM3.pin.PAD0.ABCD=reshape([3 2],1,2);MCHP.module.SERCOM3.pin.PAD1.txt=reshape({ 'PA17','PA23'},1,2);MCHP.module.SERCOM3.pin.PAD1.Rx_idx=reshape([17 23],1,2);MCHP.module.SERCOM3.pin.PAD1.ABCD=reshape([3 2],1,2);MCHP.module.SERCOM3.pin.PAD2.txt=reshape({ 'PA18','PA20','PA24'},1,3);MCHP.module.SERCOM3.pin.PAD2.Rx_idx=reshape([18 20 24],1,3);MCHP.module.SERCOM3.pin.PAD2.ABCD=reshape([3 3 2],1,3);MCHP.module.SERCOM3.pin.PAD3.txt=reshape({ 'PA19','PA21','PA25'},1,3);MCHP.module.SERCOM3.pin.PAD3.Rx_idx=reshape([19 21 25],1,3);MCHP.module.SERCOM3.pin.PAD3.ABCD=reshape([3 3 2],1,3);MCHP.module.SERCOM4.PID=13;MCHP.module.SERCOM4.vector='SERCOM4';MCHP.module.SERCOM4.pin.PAD0.txt=reshape({ 'PA12','PB08','PB12'},1,3);MCHP.module.SERCOM4.pin.PAD0.Rx_idx=reshape([12 40 44],1,3);MCHP.module.SERCOM4.pin.PAD0.ABCD=reshape([3 3 2],1,3);MCHP.module.SERCOM4.pin.PAD1.txt=reshape({ 'PA13','PB09','PB13'},1,3);MCHP.module.SERCOM4.pin.PAD1.Rx_idx=reshape([13 41 45],1,3);MCHP.module.SERCOM4.pin.PAD1.ABCD=reshape([3 3 2],1,3);MCHP.module.SERCOM4.pin.PAD2.txt=reshape({ 'PA14','PB10','PB14'},1,3);MCHP.module.SERCOM4.pin.PAD2.Rx_idx=reshape([14 42 46],1,3);MCHP.module.SERCOM4.pin.PAD2.ABCD=reshape([3 3 2],1,3);MCHP.module.SERCOM4.pin.PAD3.txt=reshape({ 'PA15','PB11','PB15'},1,3);MCHP.module.SERCOM4.pin.PAD3.Rx_idx=reshape([15 43 47],1,3);MCHP.module.SERCOM4.pin.PAD3.ABCD=reshape([3 3 2],1,3);MCHP.module.SERCOM5.PID=14;MCHP.module.SERCOM5.vector='SERCOM5';MCHP.module.SERCOM5.pin.PAD0.txt=reshape({ 'PA22','PB02','PB30','PB16'},1,4);MCHP.module.SERCOM5.pin.PAD0.Rx_idx=reshape([22 34 62 48],1,4);MCHP.module.SERCOM5.pin.PAD0.ABCD=reshape([3 3 3 2],1,4);MCHP.module.SERCOM5.pin.PAD1.txt=reshape({ 'PA23','PB03','PB31','PB17'},1,4);MCHP.module.SERCOM5.pin.PAD1.Rx_idx=reshape([23 35 63 49],1,4);MCHP.module.SERCOM5.pin.PAD1.ABCD=reshape([3 3 3 2],1,4);MCHP.module.SERCOM5.pin.PAD2.txt=reshape({ 'PA24','PB00','PB22','PA20'},1,4);MCHP.module.SERCOM5.pin.PAD2.Rx_idx=reshape([24 32 54 20],1,4);MCHP.module.SERCOM5.pin.PAD2.ABCD=reshape([3 3 3 2],1,4);MCHP.module.SERCOM5.pin.PAD3.txt=reshape({ 'PA25','PB01','PB23','PA21'},1,4);MCHP.module.SERCOM5.pin.PAD3.Rx_idx=reshape([25 33 55 21],1,4);MCHP.module.SERCOM5.pin.PAD3.ABCD=reshape([3 3 3 2],1,4);MCHP.module.CAN0.PID=15;MCHP.module.CAN0.vector='CAN0';MCHP.module.CAN0.pin.RX.txt=reshape({ 'PA25','PB23'},1,2);MCHP.module.CAN0.pin.RX.Rx_idx=reshape([25 55],1,2);MCHP.module.CAN0.pin.RX.ABCD=reshape([6 6],1,2);MCHP.module.CAN0.pin.TX.txt=reshape({ 'PA24','PB22'},1,2);MCHP.module.CAN0.pin.TX.Rx_idx=reshape([24 54],1,2);MCHP.module.CAN0.pin.TX.ABCD=reshape([6 6],1,2);MCHP.module.CAN1.PID=16;MCHP.module.CAN1.vector='CAN1';MCHP.module.CAN1.pin.RX.txt=reshape({ 'PB11','PB15'},1,2);MCHP.module.CAN1.pin.RX.Rx_idx=reshape([43 47],1,2);MCHP.module.CAN1.pin.RX.ABCD=reshape([6 6],1,2);MCHP.module.CAN1.pin.TX.txt=reshape({ 'PB10','PB14'},1,2);MCHP.module.CAN1.pin.TX.Rx_idx=reshape([42 46],1,2);MCHP.module.CAN1.pin.TX.ABCD=reshape([6 6],1,2);MCHP.module.TCC0.PID=17;MCHP.module.TCC0.vector='TCC0';MCHP.module.TCC0.pin.WO0.txt=reshape({ 'PA04','PA08','PB30'},1,3);MCHP.module.TCC0.pin.WO0.Rx_idx=reshape([4 8 62],1,3);MCHP.module.TCC0.pin.WO0.ABCD=reshape([4 4 4],1,3);MCHP.module.TCC0.pin.WO1.txt=reshape({ 'PA05','PA09','PB31'},1,3);MCHP.module.TCC0.pin.WO1.Rx_idx=reshape([5 9 63],1,3);MCHP.module.TCC0.pin.WO1.ABCD=reshape([4 4 4],1,3);MCHP.module.TCC0.pin.WO2.txt=reshape({ 'PA10','PA18'},1,2);MCHP.module.TCC0.pin.WO2.Rx_idx=reshape([10 18],1,2);MCHP.module.TCC0.pin.WO2.ABCD=reshape([5 5],1,2);MCHP.module.TCC0.pin.WO3.txt=reshape({ 'PA11','PA19'},1,2);MCHP.module.TCC0.pin.WO3.Rx_idx=reshape([11 19],1,2);MCHP.module.TCC0.pin.WO3.ABCD=reshape([5 5],1,2);MCHP.module.TCC0.pin.WO4.txt=reshape({ 'PA22','PB10','PB16','PA14'},1,4);MCHP.module.TCC0.pin.WO4.Rx_idx=reshape([22 42 48 14],1,4);MCHP.module.TCC0.pin.WO4.ABCD=reshape([5 5 5 5],1,4);MCHP.module.TCC0.pin.WO5.txt=reshape({ 'PA15','PA23','PB11','PB17'},1,4);MCHP.module.TCC0.pin.WO5.Rx_idx=reshape([15 23 43 49],1,4);MCHP.module.TCC0.pin.WO5.ABCD=reshape([5 5 5 5],1,4);MCHP.module.TCC0.pin.WO6.txt=reshape({ 'PA12','PA16','PA20','PB12'},1,4);MCHP.module.TCC0.pin.WO6.Rx_idx=reshape([12 16 20 44],1,4);MCHP.module.TCC0.pin.WO6.ABCD=reshape([5 5 5 5],1,4);MCHP.module.TCC0.pin.WO7.txt=reshape({ 'PA13','PA17','PA21','PB13'},1,4);MCHP.module.TCC0.pin.WO7.Rx_idx=reshape([13 17 21 45],1,4);MCHP.module.TCC0.pin.WO7.ABCD=reshape([5 5 5 5],1,4);MCHP.module.TCC1.PID=18;MCHP.module.TCC1.vector='TCC1';MCHP.module.TCC1.pin.WO0.txt=reshape({ 'PA06','PA10','PA30'},1,3);MCHP.module.TCC1.pin.WO0.Rx_idx=reshape([6 10 30],1,3);MCHP.module.TCC1.pin.WO0.ABCD=reshape([4 4 4],1,3);MCHP.module.TCC1.pin.WO1.txt=reshape({ 'PA07','PA11','PA31'},1,3);MCHP.module.TCC1.pin.WO1.Rx_idx=reshape([7 11 31],1,3);MCHP.module.TCC1.pin.WO1.ABCD=reshape([4 4 4],1,3);MCHP.module.TCC1.pin.WO2.txt=reshape({ 'PA08','PA24','PB30'},1,3);MCHP.module.TCC1.pin.WO2.Rx_idx=reshape([8 24 62],1,3);MCHP.module.TCC1.pin.WO2.ABCD=reshape([5 5 5],1,3);MCHP.module.TCC1.pin.WO3.txt=reshape({ 'PA09','PA25','PB31'},1,3);MCHP.module.TCC1.pin.WO3.Rx_idx=reshape([9 25 63],1,3);MCHP.module.TCC1.pin.WO3.ABCD=reshape([5 5 5],1,3);MCHP.module.TCC2.PID=19;MCHP.module.TCC2.vector='TCC2';MCHP.module.TCC2.pin.WO0.txt=reshape({ 'PA12','PA16','PA00'},1,3);MCHP.module.TCC2.pin.WO0.Rx_idx=reshape([12 16 0],1,3);MCHP.module.TCC2.pin.WO0.ABCD=reshape([4 4 4],1,3);MCHP.module.TCC2.pin.WO1.txt=reshape({ 'PA13','PA17','PA01'},1,3);MCHP.module.TCC2.pin.WO1.Rx_idx=reshape([13 17 1],1,3);MCHP.module.TCC2.pin.WO1.ABCD=reshape([4 4 4],1,3);MCHP.module.TC0.PID=20;MCHP.module.TC0.vector='TC0';MCHP.module.TC0.pin.WO0.txt=reshape({ 'PA22','PB08','PB12'},1,3);MCHP.module.TC0.pin.WO0.Rx_idx=reshape([22 40 44],1,3);MCHP.module.TC0.pin.WO0.ABCD=reshape([4 4 4],1,3);MCHP.module.TC0.pin.WO1.txt=reshape({ 'PA23','PB09','PB13'},1,3);MCHP.module.TC0.pin.WO1.Rx_idx=reshape([23 41 45],1,3);MCHP.module.TC0.pin.WO1.ABCD=reshape([4 4 4],1,3);MCHP.module.TC1.PID=21;MCHP.module.TC1.vector='TC1';MCHP.module.TC1.pin.WO0.txt=reshape({ 'PA24','PB10','PB14'},1,3);MCHP.module.TC1.pin.WO0.Rx_idx=reshape([24 42 46],1,3);MCHP.module.TC1.pin.WO0.ABCD=reshape([4 4 4],1,3);MCHP.module.TC1.pin.WO1.txt=reshape({ 'PA25','PB11','PB15'},1,3);MCHP.module.TC1.pin.WO1.Rx_idx=reshape([25 43 47],1,3);MCHP.module.TC1.pin.WO1.ABCD=reshape([4 4 4],1,3);MCHP.module.TC2.PID=22;MCHP.module.TC2.vector='TC2';MCHP.module.TC2.pin.WO0.txt=reshape({ 'PB02','PB16'},1,2);MCHP.module.TC2.pin.WO0.Rx_idx=reshape([34 48],1,2);MCHP.module.TC2.pin.WO0.ABCD=reshape([4 4],1,2);MCHP.module.TC2.pin.WO1.txt=reshape({ 'PB03','PB17'},1,2);MCHP.module.TC2.pin.WO1.Rx_idx=reshape([35 49],1,2);MCHP.module.TC2.pin.WO1.ABCD=reshape([4 4],1,2);MCHP.module.TC3.PID=23;MCHP.module.TC3.vector='TC3';MCHP.module.TC3.pin.WO0.txt=reshape({ 'PA20','PB00','PB22'},1,3);MCHP.module.TC3.pin.WO0.Rx_idx=reshape([20 32 54],1,3);MCHP.module.TC3.pin.WO0.ABCD=reshape([4 4 4],1,3);MCHP.module.TC3.pin.WO1.txt=reshape({ 'PA21','PB01','PB23'},1,3);MCHP.module.TC3.pin.WO1.Rx_idx=reshape([21 33 55],1,3);MCHP.module.TC3.pin.WO1.ABCD=reshape([4 4 4],1,3);MCHP.module.TC4.PID=24;MCHP.module.TC4.vector='TC4';MCHP.module.TC4.pin.WO0.txt=reshape({ 'PA18','PA14'},1,2);MCHP.module.TC4.pin.WO0.Rx_idx=reshape([18 14],1,2);MCHP.module.TC4.pin.WO0.ABCD=reshape([4 4],1,2);MCHP.module.TC4.pin.WO1.txt=reshape({ 'PA19','PA15'},1,2);MCHP.module.TC4.pin.WO1.Rx_idx=reshape([19 15],1,2);MCHP.module.TC4.pin.WO1.ABCD=reshape([4 4],1,2);MCHP.module.ADC0.PID=25;MCHP.module.ADC0.vector='ADC0';MCHP.module.ADC0.pin.AIN0.txt={ 'PA02'};MCHP.module.ADC0.pin.AIN0.Rx_idx=2;MCHP.module.ADC0.pin.AIN0.ABCD=1;MCHP.module.ADC0.pin.AIN1.txt={ 'PA03'};MCHP.module.ADC0.pin.AIN1.Rx_idx=3;MCHP.module.ADC0.pin.AIN1.ABCD=1;MCHP.module.ADC0.pin.AIN2.txt={ 'PB08'};MCHP.module.ADC0.pin.AIN2.Rx_idx=40;MCHP.module.ADC0.pin.AIN2.ABCD=1;MCHP.module.ADC0.pin.AIN3.txt={ 'PB09'};MCHP.module.ADC0.pin.AIN3.Rx_idx=41;MCHP.module.ADC0.pin.AIN3.ABCD=1;MCHP.module.ADC0.pin.AIN4.txt={ 'PA04'};MCHP.module.ADC0.pin.AIN4.Rx_idx=4;MCHP.module.ADC0.pin.AIN4.ABCD=1;MCHP.module.ADC0.pin.AIN5.txt={ 'PA05'};MCHP.module.ADC0.pin.AIN5.Rx_idx=5;MCHP.module.ADC0.pin.AIN5.ABCD=1;MCHP.module.ADC0.pin.AIN6.txt={ 'PA06'};MCHP.module.ADC0.pin.AIN6.Rx_idx=6;MCHP.module.ADC0.pin.AIN6.ABCD=1;MCHP.module.ADC0.pin.AIN7.txt={ 'PA07'};MCHP.module.ADC0.pin.AIN7.Rx_idx=7;MCHP.module.ADC0.pin.AIN7.ABCD=1;MCHP.module.ADC0.pin.AIN8.txt={ 'PA08'};MCHP.module.ADC0.pin.AIN8.Rx_idx=8;MCHP.module.ADC0.pin.AIN8.ABCD=1;MCHP.module.ADC0.pin.AIN9.txt={ 'PA09'};MCHP.module.ADC0.pin.AIN9.Rx_idx=9;MCHP.module.ADC0.pin.AIN9.ABCD=1;MCHP.module.ADC0.pin.AIN10.txt={ 'PA10'};MCHP.module.ADC0.pin.AIN10.Rx_idx=10;MCHP.module.ADC0.pin.AIN10.ABCD=1;MCHP.module.ADC0.pin.AIN11.txt={ 'PA11'};MCHP.module.ADC0.pin.AIN11.Rx_idx=11;MCHP.module.ADC0.pin.AIN11.ABCD=1;MCHP.module.ADC0.pin.VREFP.txt={ 'PA03'};MCHP.module.ADC0.pin.VREFP.Rx_idx=3;MCHP.module.ADC0.pin.VREFP.ABCD=1;MCHP.module.ADC1.PID=26;MCHP.module.ADC1.vector='ADC1';MCHP.module.ADC1.pin.AIN0.txt={ 'PB00'};MCHP.module.ADC1.pin.AIN0.Rx_idx=32;MCHP.module.ADC1.pin.AIN0.ABCD=1;MCHP.module.ADC1.pin.AIN1.txt={ 'PB01'};MCHP.module.ADC1.pin.AIN1.Rx_idx=33;MCHP.module.ADC1.pin.AIN1.ABCD=1;MCHP.module.ADC1.pin.AIN2.txt={ 'PB02'};MCHP.module.ADC1.pin.AIN2.Rx_idx=34;MCHP.module.ADC1.pin.AIN2.ABCD=1;MCHP.module.ADC1.pin.AIN3.txt={ 'PB03'};MCHP.module.ADC1.pin.AIN3.Rx_idx=35;MCHP.module.ADC1.pin.AIN3.ABCD=1;MCHP.module.ADC1.pin.AIN4.txt={ 'PB08'};MCHP.module.ADC1.pin.AIN4.Rx_idx=40;MCHP.module.ADC1.pin.AIN4.ABCD=1;MCHP.module.ADC1.pin.AIN5.txt={ 'PB09'};MCHP.module.ADC1.pin.AIN5.Rx_idx=41;MCHP.module.ADC1.pin.AIN5.ABCD=1;MCHP.module.ADC1.pin.AIN6.txt={ 'PB04'};MCHP.module.ADC1.pin.AIN6.Rx_idx=36;MCHP.module.ADC1.pin.AIN6.ABCD=1;MCHP.module.ADC1.pin.AIN7.txt={ 'PB05'};MCHP.module.ADC1.pin.AIN7.Rx_idx=37;MCHP.module.ADC1.pin.AIN7.ABCD=1;MCHP.module.ADC1.pin.AIN8.txt={ 'PB06'};MCHP.module.ADC1.pin.AIN8.Rx_idx=38;MCHP.module.ADC1.pin.AIN8.ABCD=1;MCHP.module.ADC1.pin.AIN9.txt={ 'PB07'};MCHP.module.ADC1.pin.AIN9.Rx_idx=39;MCHP.module.ADC1.pin.AIN9.ABCD=1;MCHP.module.ADC1.pin.AIN10.txt={ 'PA08'};MCHP.module.ADC1.pin.AIN10.Rx_idx=8;MCHP.module.ADC1.pin.AIN10.ABCD=1;MCHP.module.ADC1.pin.AIN11.txt={ 'PA09'};MCHP.module.ADC1.pin.AIN11.Rx_idx=9;MCHP.module.ADC1.pin.AIN11.ABCD=1;MCHP.module.AC.PID=27;MCHP.module.AC.vector='AC';MCHP.module.AC.pin.AIN0.txt={ 'PA04'};MCHP.module.AC.pin.AIN0.Rx_idx=4;MCHP.module.AC.pin.AIN0.ABCD=1;MCHP.module.AC.pin.AIN1.txt={ 'PA05'};MCHP.module.AC.pin.AIN1.Rx_idx=5;MCHP.module.AC.pin.AIN1.ABCD=1;MCHP.module.AC.pin.AIN2.txt={ 'PA06'};MCHP.module.AC.pin.AIN2.Rx_idx=6;MCHP.module.AC.pin.AIN2.ABCD=1;MCHP.module.AC.pin.AIN3.txt={ 'PA07'};MCHP.module.AC.pin.AIN3.Rx_idx=7;MCHP.module.AC.pin.AIN3.ABCD=1;MCHP.module.AC.pin.AIN4.txt={ 'PA02'};MCHP.module.AC.pin.AIN4.Rx_idx=2;MCHP.module.AC.pin.AIN4.ABCD=1;MCHP.module.AC.pin.AIN5.txt={ 'PA03'};MCHP.module.AC.pin.AIN5.Rx_idx=3;MCHP.module.AC.pin.AIN5.ABCD=1;MCHP.module.AC.pin.AIN6.txt={ 'PB05'};MCHP.module.AC.pin.AIN6.Rx_idx=37;MCHP.module.AC.pin.AIN6.ABCD=1;MCHP.module.AC.pin.AIN7.txt={ 'PB06'};MCHP.module.AC.pin.AIN7.Rx_idx=38;MCHP.module.AC.pin.AIN7.ABCD=1;MCHP.module.AC.pin.CMP0.txt=reshape({ 'PA12','PA18'},1,2);MCHP.module.AC.pin.CMP0.Rx_idx=reshape([12 18],1,2);MCHP.module.AC.pin.CMP0.ABCD=reshape([7 7],1,2);MCHP.module.AC.pin.CMP1.txt=reshape({ 'PA13','PA19'},1,2);MCHP.module.AC.pin.CMP1.Rx_idx=reshape([13 19],1,2);MCHP.module.AC.pin.CMP1.ABCD=reshape([7 7],1,2);MCHP.module.AC.pin.CMP2.txt=reshape({ 'PA00','PA24','PB30'},1,3);MCHP.module.AC.pin.CMP2.Rx_idx=reshape([0 24 62],1,3);MCHP.module.AC.pin.CMP2.ABCD=reshape([7 7 7],1,3);MCHP.module.AC.pin.CMP3.txt=reshape({ 'PA01','PA25','PB31'},1,3);MCHP.module.AC.pin.CMP3.Rx_idx=reshape([1 25 63],1,3);MCHP.module.AC.pin.CMP3.ABCD=reshape([7 7 7],1,3);MCHP.module.DAC.PID=28;MCHP.module.DAC.vector='DAC';MCHP.module.DAC.pin.VOUT.txt={ 'PA02'};MCHP.module.DAC.pin.VOUT.Rx_idx=2;MCHP.module.DAC.pin.VOUT.ABCD=1;MCHP.module.DAC.pin.VREFP.txt={ 'PA03'};MCHP.module.DAC.pin.VREFP.Rx_idx=3;MCHP.module.DAC.pin.VREFP.ABCD=1;MCHP.module.SDADC.PID=29;MCHP.module.SDADC.vector='SDADC';MCHP.module.SDADC.pin.INN0.txt={ 'PA06'};MCHP.module.SDADC.pin.INN0.Rx_idx=6;MCHP.module.SDADC.pin.INN0.ABCD=1;MCHP.module.SDADC.pin.INN1.txt={ 'PB08'};MCHP.module.SDADC.pin.INN1.Rx_idx=40;MCHP.module.SDADC.pin.INN1.ABCD=1;MCHP.module.SDADC.pin.INN2.txt={ 'PB06'};MCHP.module.SDADC.pin.INN2.Rx_idx=38;MCHP.module.SDADC.pin.INN2.ABCD=1;MCHP.module.SDADC.pin.INP0.txt={ 'PA07'};MCHP.module.SDADC.pin.INP0.Rx_idx=7;MCHP.module.SDADC.pin.INP0.ABCD=1;MCHP.module.SDADC.pin.INP1.txt={ 'PB09'};MCHP.module.SDADC.pin.INP1.Rx_idx=41;MCHP.module.SDADC.pin.INP1.ABCD=1;MCHP.module.SDADC.pin.INP2.txt={ 'PB07'};MCHP.module.SDADC.pin.INP2.Rx_idx=39;MCHP.module.SDADC.pin.INP2.ABCD=1;MCHP.module.SDADC.pin.VREFP.txt={ 'PA04'};MCHP.module.SDADC.pin.VREFP.Rx_idx=4;MCHP.module.SDADC.pin.VREFP.ABCD=1;MCHP.module.PTC.PID=30;MCHP.module.PTC.vector='PTC';MCHP.module.PTC.pin.X0.txt={ 'PA08'};MCHP.module.PTC.pin.X0.Rx_idx=8;MCHP.module.PTC.pin.X0.ABCD=1;MCHP.module.PTC.pin.X1.txt={ 'PA09'};MCHP.module.PTC.pin.X1.Rx_idx=9;MCHP.module.PTC.pin.X1.ABCD=1;MCHP.module.PTC.pin.X2.txt={ 'PA10'};MCHP.module.PTC.pin.X2.Rx_idx=10;MCHP.module.PTC.pin.X2.ABCD=1;MCHP.module.PTC.pin.X3.txt={ 'PA11'};MCHP.module.PTC.pin.X3.Rx_idx=11;MCHP.module.PTC.pin.X3.ABCD=1;MCHP.module.PTC.pin.X4.txt={ 'PA16'};MCHP.module.PTC.pin.X4.Rx_idx=16;MCHP.module.PTC.pin.X4.ABCD=1;MCHP.module.PTC.pin.X5.txt={ 'PA17'};MCHP.module.PTC.pin.X5.Rx_idx=17;MCHP.module.PTC.pin.X5.ABCD=1;MCHP.module.PTC.pin.X6.txt={ 'PA18'};MCHP.module.PTC.pin.X6.Rx_idx=18;MCHP.module.PTC.pin.X6.ABCD=1;MCHP.module.PTC.pin.X7.txt={ 'PA19'};MCHP.module.PTC.pin.X7.Rx_idx=19;MCHP.module.PTC.pin.X7.ABCD=1;MCHP.module.PTC.pin.X8.txt={ 'PA20'};MCHP.module.PTC.pin.X8.Rx_idx=20;MCHP.module.PTC.pin.X8.ABCD=1;MCHP.module.PTC.pin.X9.txt={ 'PA21'};MCHP.module.PTC.pin.X9.Rx_idx=21;MCHP.module.PTC.pin.X9.ABCD=1;MCHP.module.PTC.pin.X10.txt={ 'PA22'};MCHP.module.PTC.pin.X10.Rx_idx=22;MCHP.module.PTC.pin.X10.ABCD=1;MCHP.module.PTC.pin.X11.txt={ 'PA23'};MCHP.module.PTC.pin.X11.Rx_idx=23;MCHP.module.PTC.pin.X11.ABCD=1;MCHP.module.PTC.pin.X12.txt={ 'PB12'};MCHP.module.PTC.pin.X12.Rx_idx=44;MCHP.module.PTC.pin.X12.ABCD=1;MCHP.module.PTC.pin.X13.txt={ 'PB13'};MCHP.module.PTC.pin.X13.Rx_idx=45;MCHP.module.PTC.pin.X13.ABCD=1;MCHP.module.PTC.pin.X14.txt={ 'PB14'};MCHP.module.PTC.pin.X14.Rx_idx=46;MCHP.module.PTC.pin.X14.ABCD=1;MCHP.module.PTC.pin.X15.txt={ 'PB15'};MCHP.module.PTC.pin.X15.Rx_idx=47;MCHP.module.PTC.pin.X15.ABCD=1;MCHP.module.PTC.pin.Y0.txt={ 'PA02'};MCHP.module.PTC.pin.Y0.Rx_idx=2;MCHP.module.PTC.pin.Y0.ABCD=1;MCHP.module.PTC.pin.Y1.txt={ 'PA03'};MCHP.module.PTC.pin.Y1.Rx_idx=3;MCHP.module.PTC.pin.Y1.ABCD=1;MCHP.module.PTC.pin.Y2.txt={ 'PA04'};MCHP.module.PTC.pin.Y2.Rx_idx=4;MCHP.module.PTC.pin.Y2.ABCD=1;MCHP.module.PTC.pin.Y3.txt={ 'PA05'};MCHP.module.PTC.pin.Y3.Rx_idx=5;MCHP.module.PTC.pin.Y3.ABCD=1;MCHP.module.PTC.pin.Y4.txt={ 'PA06'};MCHP.module.PTC.pin.Y4.Rx_idx=6;MCHP.module.PTC.pin.Y4.ABCD=1;MCHP.module.PTC.pin.Y5.txt={ 'PA07'};MCHP.module.PTC.pin.Y5.Rx_idx=7;MCHP.module.PTC.pin.Y5.ABCD=1;MCHP.module.PTC.pin.Y6.txt={ 'PB00'};MCHP.module.PTC.pin.Y6.Rx_idx=32;MCHP.module.PTC.pin.Y6.ABCD=1;MCHP.module.PTC.pin.Y7.txt={ 'PB01'};MCHP.module.PTC.pin.Y7.Rx_idx=33;MCHP.module.PTC.pin.Y7.ABCD=1;MCHP.module.PTC.pin.Y8.txt={ 'PB02'};MCHP.module.PTC.pin.Y8.Rx_idx=34;MCHP.module.PTC.pin.Y8.ABCD=1;MCHP.module.PTC.pin.Y9.txt={ 'PB03'};MCHP.module.PTC.pin.Y9.Rx_idx=35;MCHP.module.PTC.pin.Y9.ABCD=1;MCHP.module.PTC.pin.Y10.txt={ 'PB04'};MCHP.module.PTC.pin.Y10.Rx_idx=36;MCHP.module.PTC.pin.Y10.ABCD=1;MCHP.module.PTC.pin.Y11.txt={ 'PB05'};MCHP.module.PTC.pin.Y11.Rx_idx=37;MCHP.module.PTC.pin.Y11.ABCD=1;MCHP.module.PTC.pin.Y12.txt={ 'PB06'};MCHP.module.PTC.pin.Y12.Rx_idx=38;MCHP.module.PTC.pin.Y12.ABCD=1;MCHP.module.PTC.pin.Y13.txt={ 'PB07'};MCHP.module.PTC.pin.Y13.Rx_idx=39;MCHP.module.PTC.pin.Y13.ABCD=1;MCHP.module.PTC.pin.Y14.txt={ 'PB08'};MCHP.module.PTC.pin.Y14.Rx_idx=40;MCHP.module.PTC.pin.Y14.ABCD=1;MCHP.module.PTC.pin.Y15.txt={ 'PB09'};MCHP.module.PTC.pin.Y15.Rx_idx=41;MCHP.module.PTC.pin.Y15.ABCD=1;MCHP.module.PTC.pin.Y16.txt={ 'PA08'};MCHP.module.PTC.pin.Y16.Rx_idx=8;MCHP.module.PTC.pin.Y16.ABCD=1;MCHP.module.PTC.pin.Y17.txt={ 'PA09'};MCHP.module.PTC.pin.Y17.Rx_idx=9;MCHP.module.PTC.pin.Y17.ABCD=1;MCHP.module.PTC.pin.Y18.txt={ 'PA10'};MCHP.module.PTC.pin.Y18.Rx_idx=10;MCHP.module.PTC.pin.Y18.ABCD=1;MCHP.module.PTC.pin.Y19.txt={ 'PA11'};MCHP.module.PTC.pin.Y19.Rx_idx=11;MCHP.module.PTC.pin.Y19.ABCD=1;MCHP.module.PTC.pin.Y20.txt={ 'PA16'};MCHP.module.PTC.pin.Y20.Rx_idx=16;MCHP.module.PTC.pin.Y20.ABCD=1;MCHP.module.PTC.pin.Y21.txt={ 'PA17'};MCHP.module.PTC.pin.Y21.Rx_idx=17;MCHP.module.PTC.pin.Y21.ABCD=1;MCHP.module.PTC.pin.Y22.txt={ 'PA18'};MCHP.module.PTC.pin.Y22.Rx_idx=18;MCHP.module.PTC.pin.Y22.ABCD=1;MCHP.module.PTC.pin.Y23.txt={ 'PA19'};MCHP.module.PTC.pin.Y23.Rx_idx=19;MCHP.module.PTC.pin.Y23.ABCD=1;MCHP.module.PTC.pin.Y24.txt={ 'PA20'};MCHP.module.PTC.pin.Y24.Rx_idx=20;MCHP.module.PTC.pin.Y24.ABCD=1;MCHP.module.PTC.pin.Y25.txt={ 'PA21'};MCHP.module.PTC.pin.Y25.Rx_idx=21;MCHP.module.PTC.pin.Y25.ABCD=1;MCHP.module.PTC.pin.Y26.txt={ 'PA22'};MCHP.module.PTC.pin.Y26.Rx_idx=22;MCHP.module.PTC.pin.Y26.ABCD=1;MCHP.module.PTC.pin.Y27.txt={ 'PA23'};MCHP.module.PTC.pin.Y27.Rx_idx=23;MCHP.module.PTC.pin.Y27.ABCD=1;MCHP.module.PTC.pin.Y28.txt={ 'PB12'};MCHP.module.PTC.pin.Y28.Rx_idx=44;MCHP.module.PTC.pin.Y28.ABCD=1;MCHP.module.PTC.pin.Y29.txt={ 'PB13'};MCHP.module.PTC.pin.Y29.Rx_idx=45;MCHP.module.PTC.pin.Y29.ABCD=1;MCHP.module.PTC.pin.Y30.txt={ 'PB14'};MCHP.module.PTC.pin.Y30.Rx_idx=46;MCHP.module.PTC.pin.Y30.ABCD=1;MCHP.module.PTC.pin.Y31.txt={ 'PB15'};MCHP.module.PTC.pin.Y31.Rx_idx=47;MCHP.module.PTC.pin.Y31.ABCD=1;MCHP.module.CCL.pin.IN0.txt=reshape({ 'PA04','PA16','PB22'},1,3);MCHP.module.CCL.pin.IN0.Rx_idx=reshape([4 16 54],1,3);MCHP.module.CCL.pin.IN0.ABCD=reshape([8 8 8],1,3);MCHP.module.CCL.pin.IN1.txt=reshape({ 'PA05','PA17','PB00'},1,3);MCHP.module.CCL.pin.IN1.Rx_idx=reshape([5 17 32],1,3);MCHP.module.CCL.pin.IN1.ABCD=reshape([8 8 8],1,3);MCHP.module.CCL.pin.IN2.txt=reshape({ 'PA06','PA18','PB01'},1,3);MCHP.module.CCL.pin.IN2.Rx_idx=reshape([6 18 33],1,3);MCHP.module.CCL.pin.IN2.ABCD=reshape([8 8 8],1,3);MCHP.module.CCL.pin.IN3.txt=reshape({ 'PA08','PA30'},1,2);MCHP.module.CCL.pin.IN3.Rx_idx=reshape([8 30],1,2);MCHP.module.CCL.pin.IN3.ABCD=reshape([8 8],1,2);MCHP.module.CCL.pin.IN4.txt={ 'PA09'};MCHP.module.CCL.pin.IN4.Rx_idx=9;MCHP.module.CCL.pin.IN4.ABCD=8;MCHP.module.CCL.pin.IN5.txt=reshape({ 'PA10','PB10'},1,2);MCHP.module.CCL.pin.IN5.Rx_idx=reshape([10 42],1,2);MCHP.module.CCL.pin.IN5.ABCD=reshape([8 8],1,2);MCHP.module.CCL.pin.IN6.txt=reshape({ 'PA22','PB06'},1,2);MCHP.module.CCL.pin.IN6.Rx_idx=reshape([22 38],1,2);MCHP.module.CCL.pin.IN6.ABCD=reshape([8 8],1,2);MCHP.module.CCL.pin.IN7.txt=reshape({ 'PA23','PB07'},1,2);MCHP.module.CCL.pin.IN7.Rx_idx=reshape([23 39],1,2);MCHP.module.CCL.pin.IN7.ABCD=reshape([8 8],1,2);MCHP.module.CCL.pin.IN8.txt=reshape({ 'PA24','PB08'},1,2);MCHP.module.CCL.pin.IN8.Rx_idx=reshape([24 40],1,2);MCHP.module.CCL.pin.IN8.ABCD=reshape([8 8],1,2);MCHP.module.CCL.pin.IN9.txt={ 'PB14'};MCHP.module.CCL.pin.IN9.Rx_idx=46;MCHP.module.CCL.pin.IN9.ABCD=8;MCHP.module.CCL.pin.IN10.txt={ 'PB15'};MCHP.module.CCL.pin.IN10.Rx_idx=47;MCHP.module.CCL.pin.IN10.ABCD=8;MCHP.module.CCL.pin.IN11.txt={ 'PB16'};MCHP.module.CCL.pin.IN11.Rx_idx=48;MCHP.module.CCL.pin.IN11.ABCD=8;MCHP.module.CCL.pin.OUT0.txt=reshape({ 'PA07','PA19','PB02','PB23'},1,4);MCHP.module.CCL.pin.OUT0.Rx_idx=reshape([7 19 34 55],1,4);MCHP.module.CCL.pin.OUT0.ABCD=reshape([8 8 8 8],1,4);MCHP.module.CCL.pin.OUT1.txt=reshape({ 'PA11','PA31','PB11'},1,3);MCHP.module.CCL.pin.OUT1.Rx_idx=reshape([11 31 43],1,3);MCHP.module.CCL.pin.OUT1.ABCD=reshape([8 8 8],1,3);MCHP.module.CCL.pin.OUT2.txt=reshape({ 'PA25','PB09'},1,2);MCHP.module.CCL.pin.OUT2.Rx_idx=reshape([25 41],1,2);MCHP.module.CCL.pin.OUT2.ABCD=reshape([8 8],1,2);MCHP.module.CCL.pin.OUT3.txt={ 'PB17'};MCHP.module.CCL.pin.OUT3.Rx_idx=49;MCHP.module.CCL.pin.OUT3.ABCD=8;MCHP.module.GCLK.pin.IO0.txt=reshape({ 'PB14','PB22','PA14','PA27','PA30','PA28'},1,6);MCHP.module.GCLK.pin.IO0.Rx_idx=reshape([46 54 14 27 30 28],1,6);MCHP.module.GCLK.pin.IO0.ABCD=reshape([7 7 7 7 7 7],1,6);MCHP.module.GCLK.pin.IO1.txt=reshape({ 'PB15','PB23','PA15'},1,3);MCHP.module.GCLK.pin.IO1.Rx_idx=reshape([47 55 15],1,3);MCHP.module.GCLK.pin.IO1.ABCD=reshape([7 7 7],1,3);MCHP.module.GCLK.pin.IO2.txt=reshape({ 'PB16','PA16'},1,2);MCHP.module.GCLK.pin.IO2.Rx_idx=reshape([48 16],1,2);MCHP.module.GCLK.pin.IO2.ABCD=reshape([7 7],1,2);MCHP.module.GCLK.pin.IO3.txt=reshape({ 'PA17','PB17'},1,2);MCHP.module.GCLK.pin.IO3.Rx_idx=reshape([17 49],1,2);MCHP.module.GCLK.pin.IO3.ABCD=reshape([7 7],1,2);MCHP.module.GCLK.pin.IO4.txt=reshape({ 'PA10','PA20','PB10'},1,3);MCHP.module.GCLK.pin.IO4.Rx_idx=reshape([10 20 42],1,3);MCHP.module.GCLK.pin.IO4.ABCD=reshape([7 7 7],1,3);MCHP.module.GCLK.pin.IO5.txt=reshape({ 'PA11','PA21','PB11'},1,3);MCHP.module.GCLK.pin.IO5.Rx_idx=reshape([11 21 43],1,3);MCHP.module.GCLK.pin.IO5.ABCD=reshape([7 7 7],1,3);MCHP.module.GCLK.pin.IO6.txt=reshape({ 'PA22','PB12'},1,2);MCHP.module.GCLK.pin.IO6.Rx_idx=reshape([22 44],1,2);MCHP.module.GCLK.pin.IO6.ABCD=reshape([7 7],1,2);MCHP.module.GCLK.pin.IO7.txt=reshape({ 'PA23','PB13'},1,2);MCHP.module.GCLK.pin.IO7.Rx_idx=reshape([23 45],1,2);MCHP.module.GCLK.pin.IO7.ABCD=reshape([7 7],1,2);MCHP.module.OSCCTRL.pin.XIN.txt={ 'PA14'};MCHP.module.OSCCTRL.pin.XIN.Rx_idx=14;MCHP.module.OSCCTRL.pin.XIN.ABCD=-10;MCHP.module.OSCCTRL.pin.XOSC_CLK.txt={ 'PA09'};MCHP.module.OSCCTRL.pin.XOSC_CLK.Rx_idx=9;MCHP.module.OSCCTRL.pin.XOSC_CLK.ABCD=-10;MCHP.module.OSCCTRL.pin.XOSC_EN.txt={ 'PA08'};MCHP.module.OSCCTRL.pin.XOSC_EN.Rx_idx=8;MCHP.module.OSCCTRL.pin.XOSC_EN.ABCD=-10;MCHP.module.OSCCTRL.pin.XOUT.txt={ 'PA15'};MCHP.module.OSCCTRL.pin.XOUT.Rx_idx=15;MCHP.module.OSCCTRL.pin.XOUT.ABCD=-10;MCHP.module.OSC32KCTRL.pin.XIN32.txt={ 'PA00'};MCHP.module.OSC32KCTRL.pin.XIN32.Rx_idx=0;MCHP.module.OSC32KCTRL.pin.XIN32.ABCD=-10;MCHP.module.OSC32KCTRL.pin.XOUT32.txt={ 'PA01'};MCHP.module.OSC32KCTRL.pin.XOUT32.Rx_idx=1;MCHP.module.OSC32KCTRL.pin.XOUT32.ABCD=-10;MCHP.module.RSTC.pin.EXTWAKE0.txt={ 'PA00'};MCHP.module.RSTC.pin.EXTWAKE0.Rx_idx=0;MCHP.module.RSTC.pin.EXTWAKE0.ABCD=0;MCHP.module.RSTC.pin.EXTWAKE1.txt={ 'PA01'};MCHP.module.RSTC.pin.EXTWAKE1.Rx_idx=1;MCHP.module.RSTC.pin.EXTWAKE1.ABCD=0;MCHP.module.RSTC.pin.EXTWAKE2.txt={ 'PA02'};MCHP.module.RSTC.pin.EXTWAKE2.Rx_idx=2;MCHP.module.RSTC.pin.EXTWAKE2.ABCD=0;MCHP.module.RSTC.pin.EXTWAKE3.txt={ 'PA03'};MCHP.module.RSTC.pin.EXTWAKE3.Rx_idx=3;MCHP.module.RSTC.pin.EXTWAKE3.ABCD=0;MCHP.module.RSTC.pin.EXTWAKE4.txt={ 'PA04'};MCHP.module.RSTC.pin.EXTWAKE4.Rx_idx=4;MCHP.module.RSTC.pin.EXTWAKE4.ABCD=0;MCHP.module.RSTC.pin.EXTWAKE5.txt={ 'PA05'};MCHP.module.RSTC.pin.EXTWAKE5.Rx_idx=5;MCHP.module.RSTC.pin.EXTWAKE5.ABCD=0;MCHP.module.RSTC.pin.EXTWAKE6.txt={ 'PA06'};MCHP.module.RSTC.pin.EXTWAKE6.Rx_idx=6;MCHP.module.RSTC.pin.EXTWAKE6.ABCD=0;MCHP.module.RSTC.pin.EXTWAKE7.txt={ 'PA07'};MCHP.module.RSTC.pin.EXTWAKE7.Rx_idx=7;MCHP.module.RSTC.pin.EXTWAKE7.ABCD=0;MCHP.module.RSTC.pin.EXTWAKE8.txt={ 'PA08'};MCHP.module.RSTC.pin.EXTWAKE8.Rx_idx=8;MCHP.module.RSTC.pin.EXTWAKE8.ABCD=0;MCHP.module.RSTC.pin.EXTWAKE9.txt={ 'PA09'};MCHP.module.RSTC.pin.EXTWAKE9.Rx_idx=9;MCHP.module.RSTC.pin.EXTWAKE9.ABCD=0;MCHP.module.RSTC.pin.EXTWAKE10.txt={ 'PA10'};MCHP.module.RSTC.pin.EXTWAKE10.Rx_idx=10;MCHP.module.RSTC.pin.EXTWAKE10.ABCD=0;MCHP.module.RSTC.pin.EXTWAKE11.txt={ 'PA11'};MCHP.module.RSTC.pin.EXTWAKE11.Rx_idx=11;MCHP.module.RSTC.pin.EXTWAKE11.ABCD=0;MCHP.module.RSTC.pin.EXTWAKE12.txt={ 'PA12'};MCHP.module.RSTC.pin.EXTWAKE12.Rx_idx=12;MCHP.module.RSTC.pin.EXTWAKE12.ABCD=0;MCHP.module.RSTC.pin.EXTWAKE13.txt={ 'PA13'};MCHP.module.RSTC.pin.EXTWAKE13.Rx_idx=13;MCHP.module.RSTC.pin.EXTWAKE13.ABCD=0;MCHP.module.RSTC.pin.EXTWAKE14.txt={ 'PA14'};MCHP.module.RSTC.pin.EXTWAKE14.Rx_idx=14;MCHP.module.RSTC.pin.EXTWAKE14.ABCD=0;MCHP.module.RSTC.pin.EXTWAKE15.txt={ 'PA15'};MCHP.module.RSTC.pin.EXTWAKE15.Rx_idx=15;MCHP.module.RSTC.pin.EXTWAKE15.ABCD=0;MCHP.module.SUPC.pin.BGBUFREADY0.txt={ 'PA08'};MCHP.module.SUPC.pin.BGBUFREADY0.Rx_idx=8;MCHP.module.SUPC.pin.BGBUFREADY0.ABCD=-30;MCHP.module.SUPC.pin.BGBUFREADY1.txt={ 'PA09'};MCHP.module.SUPC.pin.BGBUFREADY1.Rx_idx=9;MCHP.module.SUPC.pin.BGBUFREADY1.ABCD=-30;MCHP.module.SUPC.pin.BGBUFREADY2.txt={ 'PA10'};MCHP.module.SUPC.pin.BGBUFREADY2.Rx_idx=10;MCHP.module.SUPC.pin.BGBUFREADY2.ABCD=-30;MCHP.module.SUPC.pin.BGBUFREADY3.txt={ 'PA11'};MCHP.module.SUPC.pin.BGBUFREADY3.Rx_idx=11;MCHP.module.SUPC.pin.BGBUFREADY3.ABCD=-30;MCHP.module.SUPC.pin.BGBUFREADY4.txt={ 'PA12'};MCHP.module.SUPC.pin.BGBUFREADY4.Rx_idx=12;MCHP.module.SUPC.pin.BGBUFREADY4.ABCD=-30;MCHP.module.SUPC.pin.BGBUFREADY5.txt={ 'PA07'};MCHP.module.SUPC.pin.BGBUFREADY5.Rx_idx=7;MCHP.module.SUPC.pin.BGBUFREADY5.ABCD=-30;MCHP.module.SUPC.pin.BGBUFRRREADY.txt={ 'PA04'};MCHP.module.SUPC.pin.BGBUFRRREADY.Rx_idx=4;MCHP.module.SUPC.pin.BGBUFRRREADY.ABCD=-30;MCHP.module.SUPC.pin.BIASREADY.txt={ 'PB11'};MCHP.module.SUPC.pin.BIASREADY.Rx_idx=43;MCHP.module.SUPC.pin.BIASREADY.ABCD=-30;MCHP.module.SUPC.pin.BIAS_TEST_OUT.txt={ 'PA06'};MCHP.module.SUPC.pin.BIAS_TEST_OUT.Rx_idx=6;MCHP.module.SUPC.pin.BIAS_TEST_OUT.ABCD=-30;MCHP.module.SUPC.pin.LDO_READY.txt={ 'PB30'};MCHP.module.SUPC.pin.LDO_READY.Rx_idx=62;MCHP.module.SUPC.pin.LDO_READY.ABCD=-30;MCHP.module.SUPC.pin.ULPVREF_CLKP2.txt={ 'PB14'};MCHP.module.SUPC.pin.ULPVREF_CLKP2.Rx_idx=46;MCHP.module.SUPC.pin.ULPVREF_CLKP2.ABCD=-30;MCHP.module.SUPC.pin.VCORERDY.txt={ 'PB15'};MCHP.module.SUPC.pin.VCORERDY.Rx_idx=47;MCHP.module.SUPC.pin.VCORERDY.ABCD=-30;MCHP.module.SUPC.pin.VREFREADY0.txt={ 'PB01'};MCHP.module.SUPC.pin.VREFREADY0.Rx_idx=33;MCHP.module.SUPC.pin.VREFREADY0.ABCD=-30;MCHP.module.SUPC.pin.VREFREADY1.txt={ 'PA03'};MCHP.module.SUPC.pin.VREFREADY1.Rx_idx=3;MCHP.module.SUPC.pin.VREFREADY1.ABCD=-30;MCHP.module.SUPC.pin.VREFREADY2.txt={ 'PB31'};MCHP.module.SUPC.pin.VREFREADY2.Rx_idx=63;MCHP.module.SUPC.pin.VREFREADY2.ABCD=-30;MCHP.module.SUPC.pin.VREF_ANA_OUT.txt={ 'PA05'};MCHP.module.SUPC.pin.VREF_ANA_OUT.Rx_idx=5;MCHP.module.SUPC.pin.VREF_ANA_OUT.ABCD=-30;MCHP.module.FUSES.reglist=reshape({ 'USER_WORD_0','USER_WORD_1'},1,2);MCHP.module.FUSES.reg.USER_WORD_0.caption='USER Page Word 0';MCHP.module.FUSES.reg.USER_WORD_0.bitfieldList=reshape({ 'NVMCTRL_BOOTPROT','NVMCTRL_EEPROM_SIZE','BODVDDUSERLEVEL','BODVDD_DIS','BODVDD_ACTION','WDT_ENABLE','WDT_ALWAYSON','WDT_PER'},1,8);MCHP.module.FUSES.reg.USER_WORD_0.NVMCTRL_BOOTPROT.mask=8;MCHP.module.FUSES.reg.USER_WORD_0.NVMCTRL_BOOTPROT.choice=reshape({ 'SIZE_0BYTES','SIZE_512BYTES','SIZE_1024BYTES','SIZE_2048BYTES','SIZE_4096BYTES','SIZE_8192BYTES','SIZE_16384BYTES','SIZE_32768BYTES'},1,8);MCHP.module.FUSES.reg.USER_WORD_0.NVMCTRL_BOOTPROT.choiceCaption=reshape({ '0 Bytes','512 Bytes','1024 Bytes','2048 Bytes','4096 Bytes','8192 Bytes','16384 Bytes','32768 Bytes'},1,8);MCHP.module.FUSES.reg.USER_WORD_0.NVMCTRL_BOOTPROT.choiceDefault='SIZE_0BYTES';MCHP.module.FUSES.reg.USER_WORD_0.NVMCTRL_EEPROM_SIZE.mask=8;MCHP.module.FUSES.reg.USER_WORD_0.NVMCTRL_EEPROM_SIZE.choice=reshape({ 'SIZE_0BYTES','SIZE_256BYTES','SIZE_512BYTES','SIZE_1024BYTES','SIZE_2048BYTES','SIZE_4096BYTES','SIZE_8192BYTES','SIZE_16384BYTES'},1,8);MCHP.module.FUSES.reg.USER_WORD_0.NVMCTRL_EEPROM_SIZE.choiceCaption=reshape({ '0 Bytes','256 Bytes','512 Bytes','1024 Bytes','2048 Bytes','4096 Bytes','8192 Bytes','16384 Bytes'},1,8);MCHP.module.FUSES.reg.USER_WORD_0.NVMCTRL_EEPROM_SIZE.choiceDefault='SIZE_16384BYTES';MCHP.module.FUSES.reg.USER_WORD_0.BODVDDUSERLEVEL.mask=64;MCHP.module.FUSES.reg.USER_WORD_0.BODVDDUSERLEVEL.choice=reshape({ '0','1','2','3','4','5','6','7','8','9','A','B','C','D','E','F','10','11','12','13','14','15','16','17','18','19','1A','1B','1C','1D','1E','1F','20','21','22','23','24','25','26','27','28','29','2A','2B','2C','2D','2E','2F','30','31','32','33','34','35','36','37','38','39','3A','3B','3C','3D','3E','3F','40'},1,65);MCHP.module.FUSES.reg.USER_WORD_0.BODVDDUSERLEVEL.choiceCaption=reshape({ '0','1','2','3','4','5','6','7','8','9','A','B','C','D','E','F','10','11','12','13','14','15','16','17','18','19','1A','1B','1C','1D','1E','1F','20','21','22','23','24','25','26','27','28','29','2A','2B','2C','2D','2E','2F','30','31','32','33','34','35','36','37','38','39','3A','3B','3C','3D','3E','3F','40'},1,65);MCHP.module.FUSES.reg.USER_WORD_0.BODVDDUSERLEVEL.choiceDefault='0x3F';MCHP.module.FUSES.reg.USER_WORD_0.BODVDD_DIS.mask=2;MCHP.module.FUSES.reg.USER_WORD_0.BODVDD_DIS.choice=reshape({ 'DISABLED','ENABLED'},1,2);MCHP.module.FUSES.reg.USER_WORD_0.BODVDD_DIS.choiceCaption=reshape({ 'BODVDD is disabled','BODVDD is enabled'},1,2);MCHP.module.FUSES.reg.USER_WORD_0.BODVDD_DIS.choiceDefault='ENABLED';MCHP.module.FUSES.reg.USER_WORD_0.BODVDD_ACTION.mask=4;MCHP.module.FUSES.reg.USER_WORD_0.BODVDD_ACTION.choice=reshape({ 'NONE','RESET','INT'},1,3);MCHP.module.FUSES.reg.USER_WORD_0.BODVDD_ACTION.choiceCaption=reshape({ 'No action','The BODVDD generates a reset','The BODVDD generates an interrupt'},1,3);MCHP.module.FUSES.reg.USER_WORD_0.BODVDD_ACTION.choiceDefault='INT';MCHP.module.FUSES.reg.USER_WORD_0.WDT_ENABLE.mask=2;MCHP.module.FUSES.reg.USER_WORD_0.WDT_ENABLE.choice=reshape({ 'DISABLED','ENABLED'},1,2);MCHP.module.FUSES.reg.USER_WORD_0.WDT_ENABLE.choiceCaption=reshape({ 'WDT is disabled','WDT is enabled'},1,2);MCHP.module.FUSES.reg.USER_WORD_0.WDT_ENABLE.choiceDefault='DISABLED';MCHP.module.FUSES.reg.USER_WORD_0.WDT_ALWAYSON.mask=2;MCHP.module.FUSES.reg.USER_WORD_0.WDT_ALWAYSON.choice=reshape({ 'DISABLED','ENABLED'},1,2);MCHP.module.FUSES.reg.USER_WORD_0.WDT_ALWAYSON.choiceCaption=reshape({ 'WDT is enabled and disabled through ENABLE bit','WDT is enabled and can only be disabled by a power-on reset'},1,2);MCHP.module.FUSES.reg.USER_WORD_0.WDT_ALWAYSON.choiceDefault='DISABLED';MCHP.module.FUSES.reg.USER_WORD_0.WDT_PER.mask=16;MCHP.module.FUSES.reg.USER_WORD_0.WDT_PER.choice=reshape({ 'CYC8','CYC16','CYC32','CYC64','CYC128','CYC256','CYC512','CYC1024','CYC2048','CYC4096','CYC8192','CYC16384'},1,12);MCHP.module.FUSES.reg.USER_WORD_0.WDT_PER.choiceCaption=reshape({ '8 clock cycles','16 clock cycles','32 clock cycles','64 clock cycles','128 clock cycles','256 clock cycles','512 clock cycles','1024 clock cycles','2048 clock cycles','4096 clock cycles','8192 clock cycles','16384 clock cycles'},1,12);MCHP.module.FUSES.reg.USER_WORD_0.WDT_PER.choiceDefault='CYC16384';MCHP.module.FUSES.reg.USER_WORD_1.caption='USER Page Word 1';MCHP.module.FUSES.reg.USER_WORD_1.bitfieldList=reshape({ 'WDT_WINDOW','WDT_EWOFFSET','WDT_WEN','BODVDD_HYST','NVMCTRL_REGION_LOCKS'},1,5);MCHP.module.FUSES.reg.USER_WORD_1.WDT_WINDOW.mask=16;MCHP.module.FUSES.reg.USER_WORD_1.WDT_WINDOW.choice=reshape({ 'CYC8','CYC16','CYC32','CYC64','CYC128','CYC256','CYC512','CYC1024','CYC2048','CYC4096','CYC8192','CYC16384'},1,12);MCHP.module.FUSES.reg.USER_WORD_1.WDT_WINDOW.choiceCaption=reshape({ '8 clock cycles','16 clock cycles','32 clock cycles','64 clock cycles','128 clock cycles','256 clock cycles','512 clock cycles','1024 clock cycles','2048 clock cycles','4096 clock cycles','8192 clock cycles','16384 clock cycles'},1,12);MCHP.module.FUSES.reg.USER_WORD_1.WDT_WINDOW.choiceDefault='CYC16384';MCHP.module.FUSES.reg.USER_WORD_1.WDT_EWOFFSET.mask=16;MCHP.module.FUSES.reg.USER_WORD_1.WDT_EWOFFSET.choice=reshape({ 'CYC8','CYC16','CYC32','CYC64','CYC128','CYC256','CYC512','CYC1024','CYC2048','CYC4096','CYC8192','CYC16384'},1,12);MCHP.module.FUSES.reg.USER_WORD_1.WDT_EWOFFSET.choiceCaption=reshape({ '8 clock cycles','16 clock cycles','32 clock cycles','64 clock cycles','128 clock cycles','256 clock cycles','512 clock cycles','1024 clock cycles','2048 clock cycles','4096 clock cycles','8192 clock cycles','16384 clock cycles'},1,12);MCHP.module.FUSES.reg.USER_WORD_1.WDT_EWOFFSET.choiceDefault='CYC16384';MCHP.module.FUSES.reg.USER_WORD_1.WDT_WEN.mask=2;MCHP.module.FUSES.reg.USER_WORD_1.WDT_WEN.choice=reshape({ 'DISABLED','ENABLED'},1,2);MCHP.module.FUSES.reg.USER_WORD_1.WDT_WEN.choiceCaption=reshape({ 'WDT is disabled','WDT is enabled'},1,2);MCHP.module.FUSES.reg.USER_WORD_1.WDT_WEN.choiceDefault='DISABLED';MCHP.module.FUSES.reg.USER_WORD_1.BODVDD_HYST.mask=2;MCHP.module.FUSES.reg.USER_WORD_1.BODVDD_HYST.choice=reshape({ 'DISABLED','ENABLED'},1,2);MCHP.module.FUSES.reg.USER_WORD_1.BODVDD_HYST.choiceCaption=reshape({ 'No Hysteresis','Hysteresis Enabled'},1,2);MCHP.module.FUSES.reg.USER_WORD_1.BODVDD_HYST.choiceDefault='ENABLED';MCHP.module.FUSES.reg.USER_WORD_1.NVMCTRL_REGION_LOCKS.mask=65536;MCHP.module.FUSES.reg.USER_WORD_1.NVMCTRL_REGION_LOCKS.choice={};MCHP.module.FUSES.reg.USER_WORD_1.NVMCTRL_REGION_LOCKS.choiceCaption={ 'range in [0 - 65535]'};MCHP.module.FUSES.reg.USER_WORD_1.NVMCTRL_REGION_LOCKS.choiceDefault='0xFFFF';MCHP.modsrc.id_U2245=1;MCHP.modsrc.id_U2247=2;MCHP.modsrc.id_U2003=2;MCHP.modsrc.id_U2225=1;MCHP.modsrc.id_U2214=1;MCHP.modsrc.id_U2258=1;MCHP.modsrc.id_U2223=1;MCHP.modsrc.id_U2209=1;MCHP.modsrc.id_U2254=1;MCHP.modsrc.id_U2256=1;MCHP.modsrc.id_U2257=1;MCHP.modsrc.id_U2122=1;MCHP.modsrc.id_I7638=1;MCHP.modsrc.id_U2234=1;MCHP.modsrc.id_U2002=1;MCHP.modsrc.id_U2207=1;MCHP.modsrc.id_U2119=1;MCHP.modsrc.id_U2246=1;MCHP.modsrc.id_U2120=1;MCHP.modsrc.id_U2240=1;MCHP.modsrc.id_U2210=1;MCHP.modsrc.id_U2215=1;MCHP.modsrc.id_U2239=1;MCHP.modsrc.id_U2250=1;MCHP.modsrc.id_U2260=1;MCHP.modsrc.id_U2201=6;MCHP.modsrc.id_U2117=1;MCHP.modsrc.id_U2249=5;MCHP.modsrc.id_U2213=3;MCHP.modsrc.id_U2261=1;MCHP.modsrc.id_U2251=1;MCHP.modsrc.id_MPU=1;MCHP.modsrc.id_NVIC=1;MCHP.modsrc.id_SysTick=1;MCHP.modsrc.id_SystemControl=1;MCHP.modsrc_id.id_U2245.n=1;MCHP.modsrc_id.id_U2245.name='AC';MCHP.modsrc_id.id_U2245.version='1.1.1';MCHP.modsrc_id.id_U2247.n=2;MCHP.modsrc_id.id_U2247.name='ADC';MCHP.modsrc_id.id_U2247.version='2.2.0';MCHP.modsrc_id.id_U2003.n=2;MCHP.modsrc_id.id_U2003.name='CAN';MCHP.modsrc_id.id_U2003.version='2.0.0';MCHP.modsrc_id.id_U2225.n=1;MCHP.modsrc_id.id_U2225.name='CCL';MCHP.modsrc_id.id_U2225.version='1.0.1';MCHP.modsrc_id.id_U2214.n=1;MCHP.modsrc_id.id_U2214.name='DAC';MCHP.modsrc_id.id_U2214.version='2.0.1';MCHP.modsrc_id.id_U2258.n=1;MCHP.modsrc_id.id_U2258.name='DIVAS';MCHP.modsrc_id.id_U2258.version='1.0.0';MCHP.modsrc_id.id_U2223.n=1;MCHP.modsrc_id.id_U2223.name='DMAC';MCHP.modsrc_id.id_U2223.version='2.2.3';MCHP.modsrc_id.id_U2209.n=1;MCHP.modsrc_id.id_U2209.name='DSU';MCHP.modsrc_id.id_U2209.version='2.5.0';MCHP.modsrc_id.id_U2254.n=1;MCHP.modsrc_id.id_U2254.name='EIC';MCHP.modsrc_id.id_U2254.version='2.0.4';MCHP.modsrc_id.id_U2256.n=1;MCHP.modsrc_id.id_U2256.name='EVSYS';MCHP.modsrc_id.id_U2256.version='1.0.2';MCHP.modsrc_id.id_U2257.n=1;MCHP.modsrc_id.id_U2257.name='FREQM';MCHP.modsrc_id.id_U2257.version='1.0.1';MCHP.modsrc_id.id_U2122.n=1;MCHP.modsrc_id.id_U2122.name='GCLK';MCHP.modsrc_id.id_U2122.version='1.1.1';MCHP.modsrc_id.id_I7638.n=1;MCHP.modsrc_id.id_I7638.name='HMATRIXB';MCHP.modsrc_id.id_I7638.version='2.1.3';MCHP.modsrc_id.id_U2234.n=1;MCHP.modsrc_id.id_U2234.name='MCLK';MCHP.modsrc_id.id_U2234.version='2.0.0';MCHP.modsrc_id.id_U2002.n=1;MCHP.modsrc_id.id_U2002.name='MTB';MCHP.modsrc_id.id_U2002.version='1.0.0';MCHP.modsrc_id.id_U2207.n=1;MCHP.modsrc_id.id_U2207.name='FUSES';MCHP.modsrc_id.id_U2207.version='4.0.1.1';MCHP.modsrc_id.id_U2119.n=1;MCHP.modsrc_id.id_U2119.name='OSCCTRL';MCHP.modsrc_id.id_U2119.version='2.1.0';MCHP.modsrc_id.id_U2246.n=1;MCHP.modsrc_id.id_U2246.name='OSC32KCTRL';MCHP.modsrc_id.id_U2246.version='2.1.0';MCHP.modsrc_id.id_U2120.n=1;MCHP.modsrc_id.id_U2120.name='PAC';MCHP.modsrc_id.id_U2120.version='1.1.0';MCHP.modsrc_id.id_U2240.n=1;MCHP.modsrc_id.id_U2240.name='PM';MCHP.modsrc_id.id_U2240.version='2.1.0';MCHP.modsrc_id.id_U2210.n=1;MCHP.modsrc_id.id_U2210.name='PORT';MCHP.modsrc_id.id_U2210.version='2.1.1';MCHP.modsrc_id.id_U2215.n=1;MCHP.modsrc_id.id_U2215.name='PTC';MCHP.modsrc_id.id_U2215.version='3.1.0';MCHP.modsrc_id.id_U2239.n=1;MCHP.modsrc_id.id_U2239.name='RSTC';MCHP.modsrc_id.id_U2239.version='2.0.2';MCHP.modsrc_id.id_U2250.n=1;MCHP.modsrc_id.id_U2250.name='RTC';MCHP.modsrc_id.id_U2250.version='1.1.1';MCHP.modsrc_id.id_U2260.n=1;MCHP.modsrc_id.id_U2260.name='SDADC';MCHP.modsrc_id.id_U2260.version='1.0.1';MCHP.modsrc_id.id_U2201.n=6;MCHP.modsrc_id.id_U2201.name='SERCOM';MCHP.modsrc_id.id_U2201.version='3.1.1';MCHP.modsrc_id.id_U2117.n=1;MCHP.modsrc_id.id_U2117.name='SUPC';MCHP.modsrc_id.id_U2117.version='2.1.1';MCHP.modsrc_id.id_U2249.n=5;MCHP.modsrc_id.id_U2249.name='TC';MCHP.modsrc_id.id_U2249.version='2.0.0';MCHP.modsrc_id.id_U2213.n=3;MCHP.modsrc_id.id_U2213.name='TCC';MCHP.modsrc_id.id_U2213.version='3.0.0';MCHP.modsrc_id.id_U2261.n=1;MCHP.modsrc_id.id_U2261.name='TSENS';MCHP.modsrc_id.id_U2261.version='1.0.1';MCHP.modsrc_id.id_U2251.n=1;MCHP.modsrc_id.id_U2251.name='WDT';MCHP.modsrc_id.id_U2251.version='1.0.1';MCHP.modsrc_id.id_MPU.n=1;MCHP.modsrc_id.id_MPU.name='MPU';MCHP.modsrc_id.id_MPU.version='1.0.0';MCHP.modsrc_id.id_NVIC.n=1;MCHP.modsrc_id.id_NVIC.name='NVIC';MCHP.modsrc_id.id_NVIC.version='1.0.0';MCHP.modsrc_id.id_SysTick.n=1;MCHP.modsrc_id.id_SysTick.name='SysTick';MCHP.modsrc_id.id_SysTick.version='1.0.0';MCHP.modsrc_id.id_SystemControl.n=1;MCHP.modsrc_id.id_SystemControl.name='SystemControl';MCHP.modsrc_id.id_SystemControl.version='1.0.0';MCHP.modsrc_Name.AC.n=1;MCHP.modsrc_Name.AC.id='U2245';MCHP.modsrc_Name.AC.version='1.1.1';MCHP.modsrc_Name.ADC.n=2;MCHP.modsrc_Name.ADC.id='U2247';MCHP.modsrc_Name.ADC.version='2.2.0';MCHP.modsrc_Name.CAN.n=2;MCHP.modsrc_Name.CAN.id='U2003';MCHP.modsrc_Name.CAN.version='2.0.0';MCHP.modsrc_Name.CCL.n=1;MCHP.modsrc_Name.CCL.id='U2225';MCHP.modsrc_Name.CCL.version='1.0.1';MCHP.modsrc_Name.DAC.n=1;MCHP.modsrc_Name.DAC.id='U2214';MCHP.modsrc_Name.DAC.version='2.0.1';MCHP.modsrc_Name.DIVAS.n=1;MCHP.modsrc_Name.DIVAS.id='U2258';MCHP.modsrc_Name.DIVAS.version='1.0.0';MCHP.modsrc_Name.DMAC.n=1;MCHP.modsrc_Name.DMAC.id='U2223';MCHP.modsrc_Name.DMAC.version='2.2.3';MCHP.modsrc_Name.DSU.n=1;MCHP.modsrc_Name.DSU.id='U2209';MCHP.modsrc_Name.DSU.version='2.5.0';MCHP.modsrc_Name.EIC.n=1;MCHP.modsrc_Name.EIC.id='U2254';MCHP.modsrc_Name.EIC.version='2.0.4';MCHP.modsrc_Name.EVSYS.n=1;MCHP.modsrc_Name.EVSYS.id='U2256';MCHP.modsrc_Name.EVSYS.version='1.0.2';MCHP.modsrc_Name.FREQM.n=1;MCHP.modsrc_Name.FREQM.id='U2257';MCHP.modsrc_Name.FREQM.version='1.0.1';MCHP.modsrc_Name.GCLK.n=1;MCHP.modsrc_Name.GCLK.id='U2122';MCHP.modsrc_Name.GCLK.version='1.1.1';MCHP.modsrc_Name.HMATRIXB.n=1;MCHP.modsrc_Name.HMATRIXB.id='I7638';MCHP.modsrc_Name.HMATRIXB.version='2.1.3';MCHP.modsrc_Name.MCLK.n=1;MCHP.modsrc_Name.MCLK.id='U2234';MCHP.modsrc_Name.MCLK.version='2.0.0';MCHP.modsrc_Name.MTB.n=1;MCHP.modsrc_Name.MTB.id='U2002';MCHP.modsrc_Name.MTB.version='1.0.0';MCHP.modsrc_Name.NVMCTRL.n=1;MCHP.modsrc_Name.NVMCTRL.id='U2207';MCHP.modsrc_Name.NVMCTRL.version='4.0.1.1';MCHP.modsrc_Name.FUSES.n=1;MCHP.modsrc_Name.FUSES.id='U2207';MCHP.modsrc_Name.FUSES.version='4.0.1.1';MCHP.modsrc_Name.OSCCTRL.n=1;MCHP.modsrc_Name.OSCCTRL.id='U2119';MCHP.modsrc_Name.OSCCTRL.version='2.1.0';MCHP.modsrc_Name.OSC32KCTRL.n=1;MCHP.modsrc_Name.OSC32KCTRL.id='U2246';MCHP.modsrc_Name.OSC32KCTRL.version='2.1.0';MCHP.modsrc_Name.PAC.n=1;MCHP.modsrc_Name.PAC.id='U2120';MCHP.modsrc_Name.PAC.version='1.1.0';MCHP.modsrc_Name.PM.n=1;MCHP.modsrc_Name.PM.id='U2240';MCHP.modsrc_Name.PM.version='2.1.0';MCHP.modsrc_Name.PORT.n=1;MCHP.modsrc_Name.PORT.id='U2210';MCHP.modsrc_Name.PORT.version='2.1.1';MCHP.modsrc_Name.PTC.n=1;MCHP.modsrc_Name.PTC.id='U2215';MCHP.modsrc_Name.PTC.version='3.1.0';MCHP.modsrc_Name.RSTC.n=1;MCHP.modsrc_Name.RSTC.id='U2239';MCHP.modsrc_Name.RSTC.version='2.0.2';MCHP.modsrc_Name.RTC.n=1;MCHP.modsrc_Name.RTC.id='U2250';MCHP.modsrc_Name.RTC.version='1.1.1';MCHP.modsrc_Name.SDADC.n=1;MCHP.modsrc_Name.SDADC.id='U2260';MCHP.modsrc_Name.SDADC.version='1.0.1';MCHP.modsrc_Name.SERCOM.n=6;MCHP.modsrc_Name.SERCOM.id='U2201';MCHP.modsrc_Name.SERCOM.version='3.1.1';MCHP.modsrc_Name.SUPC.n=1;MCHP.modsrc_Name.SUPC.id='U2117';MCHP.modsrc_Name.SUPC.version='2.1.1';MCHP.modsrc_Name.TC.n=5;MCHP.modsrc_Name.TC.id='U2249';MCHP.modsrc_Name.TC.version='2.0.0';MCHP.modsrc_Name.TCC.n=3;MCHP.modsrc_Name.TCC.id='U2213';MCHP.modsrc_Name.TCC.version='3.0.0';MCHP.modsrc_Name.TSENS.n=1;MCHP.modsrc_Name.TSENS.id='U2261';MCHP.modsrc_Name.TSENS.version='1.0.1';MCHP.modsrc_Name.WDT.n=1;MCHP.modsrc_Name.WDT.id='U2251';MCHP.modsrc_Name.WDT.version='1.0.1';MCHP.modsrc_Name.MPU.n=1;MCHP.modsrc_Name.MPU.id='MPU';MCHP.modsrc_Name.MPU.version='1.0.0';MCHP.modsrc_Name.NVIC.n=1;MCHP.modsrc_Name.NVIC.id='NVIC';MCHP.modsrc_Name.NVIC.version='1.0.0';MCHP.modsrc_Name.SysTick.n=1;MCHP.modsrc_Name.SysTick.id='SysTick';MCHP.modsrc_Name.SysTick.version='1.0.0';MCHP.modsrc_Name.SystemControl.n=1;MCHP.modsrc_Name.SystemControl.id='SystemControl';MCHP.modsrc_Name.SystemControl.version='1.0.0';MCHP.PortBase=32;MCHP.PortPrefixe='P';MCHP.PowerSave=0;MCHP.fcy.GCLKx=reshape([48000000 -1 -1 -1 -1 -1 -1 -1 -1 -1 -1 -1],1,12);MCHP.fcy.MIPS=48000000;MCHP.fcy.APB_HS=48000000;MCHP.fcy.APB_CPU=48000000;MCHP.fcy.AHB_CPU=48000000;MCHP.NTIMERS=5;MCHP.SCCP.nSCCP=0;MCHP.SYS_TICK_TS_Load=47999;MCHP.TimeStepFactor=1;MCHP.INT_PRIORITY_DMA='0';  MCHP_CRC=33938899  BTMODE=Device is in Single Boot (legacy) mode  RES1=Not used  PLLSS=Not used  RES2=Not used  ALTCMPI=Not used  BOREN1=Not used  ALTRB6=Not used  RETCFG=Not used  DFMCY=Not used  BSS2=No Boot Segment  BSEN=No Boot Segment  CWRP=Configuration Segment may be written  CSS=No Protection (other than CWRP)  AIVTDIS=Disable Alternate Vector Table  BSLIM=Not used  WDTEN=Disable  BTSWP=BOOTSWP instruction is disabled  DBCC=No Cross Connection between DAC outputs  CTXT1=Not Assigned  CTXT2=Not Assigned  SEQNUM=Not used  nSEQNUM=Not used  BOREN0=Enabled  DMTIVT=Not used  DMTCNT=2^8 (256)  DMTEN=Dead Man Timer is Disabled and can be enabled by software  ON=Not used  USERID=Not used  RESERVED1=Not used  PGL1WAY=Allow only one reconfiguration  FPLLRNG=34-68 MHz Input  FPLLICLK=FRC is input to the System PLL  FPLLMULT=PLL Multiply by 128  UPLLFSEL=USB PLL input is 24 MHz  DMTINTV=Window/Interval value is 127/128 counter value  WDTSPGM=WDT stops during Flash programming  FDMTEN=Deadman Timer is disabled  TRCEN=Trace features in the CPU are enabled  BOOTISA=Boot code and Exception code is MIPS32  FECCCON=ECC and Dynamic ECC are disabled (ECCCON bits are writable)  EXTDDRSIZE=Not used  FSLEEP=Flash is powered down when the device is in Sleep mode  DBGPER=Allow CPU access to all permission regions  EJTAGBEN=Normal EJTAG functionality  TSEQ=Not used  CSEQ=Not used  RWDTPS=1:2147483648  RCLKSEL=Always use LPRC  SWDTPS=1:2147483648  DMTIVTL=Not used  DMTIVTH=Not used  DMTCNTL=Not used  DMTCNTH=Not used  DMTDIS=Dead Man Timer is Disabled and can be enabled by software  SMBEN=SMBus input threshold is enabled  SPI2PIN=SPI2 uses I/O remap (PPS) pins  CTXT3=Not Assigned  CTXT4=Not Assigned  MBXM0=Mailbox register configured for Main data read (Secondary to Main data transfer)  MBXM1=Mailbox register configured for Main data read (Secondary to Main data transfer)  MBXM2=Mailbox register configured for Main data read (Secondary to Main data transfer)  MBXM3=Mailbox register configured for Main data read (Secondary to Main data transfer)  MBXM4=Mailbox register configured for Main data read (Secondary to Main data transfer)  MBXM5=Mailbox register configured for Main data read (Secondary to Main data transfer)  MBXM6=Mailbox register configured for Main data read (Secondary to Main data transfer)  MBXM7=Mailbox register configured for Main data read (Secondary to Main data transfer)  MBXM8=Mailbox register configured for Main data read (Secondary to Main data transfer)  MBXM9=Mailbox register configured for Main data read (Secondary to Main data transfer)  MBXM10=Mailbox register configured for Main data read (Secondary to Main data transfer)  MBXM11=Mailbox register configured for Main data read (Secondary to Main data transfer)  MBXM12=Mailbox register configured for Main data read (Secondary to Main data transfer)  MBXM13=Mailbox register configured for Main data read (Secondary to Main data transfer)  MBXM14=Mailbox register configured for Main data read (Secondary to Main data transfer)  MBXM15=Mailbox register configured for Main data read (Secondary to Main data transfer)  MBXHSA=MSIxMBXD15 assigned to mailbox handshake protocol block A  MBXHSB=MSIxMBXD15 assigned to mailbox handshake protocol block B  MBXHSC=MSIxMBXD15 assigned to mailbox handshake protocol block C  MBXHSD=MSIxMBXD15 assigned to mailbox handshake protocol block D  MBXHSE=MSIxMBXD15 assigned to mailbox handshake protocol block E  MBXHSF=MSIxMBXD15 assigned to mailbox handshake protocol block F  MBXHSG=MSIxMBXD15 assigned to mailbox handshake protocol block G  MBXHSH=MSIxMBXD15 assigned to mailbox handshake protocol block H  HSAEN=Mailbox data flow control handshake protocol block disabled  HSBEN=Mailbox data flow control handshake protocol block disabled  HSCEN=Mailbox data flow control handshake protocol block disabled  HSDEN=Mailbox data flow control handshake protocol block disabled  HSEEN=Mailbox data flow control handshake protocol block disabled  HSFEN=Mailbox data flow control handshake protocol block disabled  HSGEN=Mailbox data flow control handshake protocol block disabled  HSHEN=Mailbox data flow control handshake protocol block disabled  CPRA0=Main core owns pin  CPRA1=Main core owns pin  CPRA2=Main core owns pin  CPRA3=Main core owns pin  CPRA4=Main core owns pin  CPRB0=Main core owns pin  CPRB1=Main core owns pin  CPRB2=Main core owns pin  CPRB3=Main core owns pin  CPRB4=Main core owns pin  CPRB5=Main core owns pin  CPRB6=Main core owns pin  CPRB7=Main core owns pin  CPRB8=Main core owns pin  CPRB9=Main core owns pin  CPRB10=Main core owns pin  CPRB11=Main core owns pin  CPRB12=Main core owns pin  CPRB13=Main core owns pin  CPRB14=Main core owns pin  CPRB15=Main core owns pin  CPRC0=Main core owns pin  CPRC1=Main core owns pin  CPRC2=Main core owns pin  CPRC3=Main core owns pin  CPRC4=Main core owns pin  CPRC5=Main core owns pin  CPRC6=Main core owns pin  CPRC7=Main core owns pin  CPRC8=Main core owns pin  CPRC9=Main core owns pin  CPRC10=Main core owns pin  CPRC11=Main core owns pin  CPRC12=Main core owns pin  CPRC13=Main core owns pin  CPRC14=Main core owns pin  CPRC15=Main core owns pin  CPRD0=Main core owns pin  CPRD1=Main core owns pin  CPRD2=Main core owns pin  CPRD3=Main core owns pin  CPRD4=Main core owns pin  CPRD5=Main core owns pin  CPRD6=Main core owns pin  CPRD7=Main core owns pin  CPRD8=Main core owns pin  CPRD9=Main core owns pin  CPRD10=Main core owns pin  CPRD11=Main core owns pin  CPRD12=Main core owns pin  CPRD13=Main core owns pin  CPRD14=Main core owns pin  CPRD15=Main core owns pin  CPRE0=Main core owns pin  CPRE1=Main core owns pin  CPRE2=Main core owns pin  CPRE3=Main core owns pin  CPRE4=Main core owns pin  CPRE5=Main core owns pin  CPRE6=Main core owns pin  CPRE7=Main core owns pin  CPRE8=Main core owns pin  CPRE9=Main core owns pin  CPRE10=Main core owns pin  CPRE11=Main core owns pin  CPRE12=Main core owns pin  CPRE13=Main core owns pin  CPRE14=Main core owns pin  CPRE15=Main core owns pin  S1FNOSC=Internal Fast RC (FRC) Oscillator with postscaler  S1IESO=Start up with FRC; then switch  S1OSCIOFNC=general purpose digital I/O pin  S1FCKSM=Both Clock switching and Fail-safe Clock Monitor are disabled  S1PLLKEN=S1PLLKEN_ON  S1RWDTPS=1:1048576  S1RCLKSEL=Always use LPRC  S1WINDIS=Watchdog Timer operates in Non-Window mode  S1WDTWIN=WDT Window is 25% of WDT period  S1SWDTPS=1:1048576  S1FWDTEN=use WDTCON.ON bit  S1ICS=Communicate on PGC1 and PGD1  S1DEBUG=Not used  S1ISOLAT=The Secondary can operate (in debug mode) even if the SLVEN bit in the MSI is zero  S1NOBTSWP=BOOTSWP instruction is disabled  S1ALTI2C1=I2C1 mapped to SDA1/SCL1 pins  S1SPI1PIN=Secondary SPI1 uses I/O remap (PPS) pins  S1SSRE=Secondary generated resets will reset the Secondary Enable Bit in the MSI module  S1MSRE=The Main software oriented RESET events (RESET Op-Code; Watchdog timeout; TRAP reset; illegalInstruction) will also cause the Secondary subsystem to reset  S1CTXT1=Not Assigned  S1CTXT2=Not Assigned  S1CTXT3=Not Assigned  S1CTXT4=Not Assigned  BORLVL=Not used  BSSO=Not used  MCA=Not used  MAXTEMP=Not used  CFGAN14=Not used  CFGAN15=Not used  S1IOL1WAY=Not used  S1BSSO=Not used  S1BACKBUG=Not used  BISTDIS=mBIST on reset feature disabled  NOBTSWP=BOOTSWP instruction is disabled  S1BISTDIS=Secondary BIST on reset feature disabled  S1DMTIVTL=Not used  S1DMTIVTH=Not used  S1DMTCNTL=Not used  S1DMTCNTH=Not used  S1DMTDIS=Secondary Dead Man Timer is Disabled and can be enabled by software  BSEQ=Not used  IBSEQ=Not used  SMB3EN=SMBus 3.0 input levels  FUSBIDIO2=USBID pin is controlled by the USB2 module  FVBUSIO2=VBUSON pin is controlled by the USB2 module  FUSBIDIO1=USBID pin is controlled by the USB1 module  FVBUSIO1=VBUSON pin is controlled by the USB1 module  VBATBOREN=Disable ZPBOR during VBAT Mode  FDSEN=Enable DSEN bit in DSCON  BORSEL=BOR trip voltage 2.1v (Non-OPAMP deviced operation)  POSCFGAIN=Gain is G3  POSCAGCDLY=Settling time = 25ms x AGCRNG  POSCAGCRNG=Range 1x  POSCAGC=Automatic Gain Control for Oscillator  FDBGWP=Not used
      settings: SourceProductName=MPLAB Device Blocks for Simulink
  wires:
  Data Type Conversion/1 -> Digital Output Write/1
  Constant/1 -> Data Type Conversion/1
